simulink model "architecture1_copy"  (R2019b)
settings: Solver=VariableStepAuto  StartTime=0.0  StopTime=25000  RelTol=1e-3
undefined symbols (not defined in the file or in its folder): t_vect
libraries: xbsIndex_r4 x1103
settings Model: Creator=s4533087  LastModifiedBy=s4533087

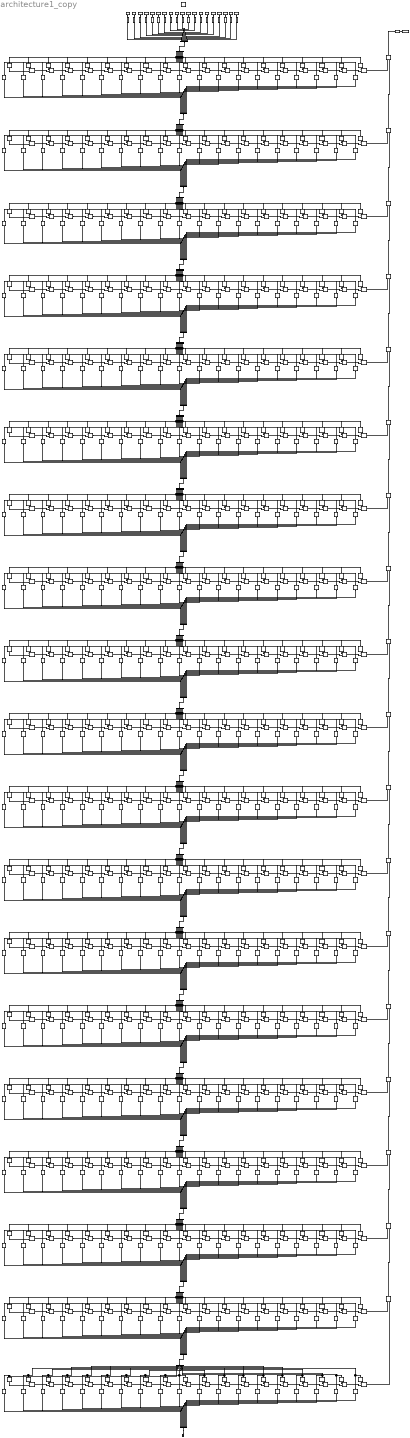
== system architecture1_copy ==
  note: Subsystem18
  note: Subsystem17
  note: Subsystem16
  note: Subsystem15
  note: Subsystem14
  note: Subsystem13
  note: Subsystem12
  note: Subsystem11
  note: Subsystem10
  note: Subsystem9
  note: Subsystem8
  note: Subsystem7
  note: Subsystem6
  note: Subsystem5
  note: Subsystem4
  note: Subsystem3
  note: Subsystem2
  note: Subsystem1
  note: Subsystem
  " System Generator" : xbsIndex_r4/ System Generator  Tag=genX  xilinxfamily=virtex7  part=xc7v2000t  speed=-1  package=flg1925  synthesis_tool=Vivado  clock_wrapper=Clock Enables  directory=./netlist  proj_type=Vivado  Synth_file=Vivado Synthesis Defaults  Impl_file=Vivado Implementation Defaults  testbench=off  simulink_period=1  sysclk_period=10  dcm_input_clock_period=10  incr_netlist=off  trim_vbits=Everywhere in SubSystem  dbl_ovrd=According to Block Masks  core_generation=According to Block Masks  run_coregen=off  deprecated_control=off  eval_field=0  block_type=sysgen
  AddSub{1..353,367,401,410,458,522,565,602} (360 alike) : xbsIndex_r4/AddSub  mode=Addition  use_carryin=off  use_carryout=off  en=off  latency=0  precision=Full  arith_type=Unsigned  n_bits=16  bin_pt=14  quantization=Truncate  overflow=Wrap  use_behavioral_HDL=off  hw_selection=Fabric  pipelined=off  dbl_ovrd=off  block_type=addsub
  Bus Creator{,1..19} (20 alike) : BusCreator  Inputs=19
  Bus Selector{,1..18} (19 alike) : BusSelector  OutputSignals=signal1,signal2,signal3,signal4,signal5,signal6,signal7,signal8,signal9,signal10,signal11,signal12,signal13,signal14,signal15,signal16,signal17,signal18,signal19
  CMult{,1,20,40,59,79,98,118,137,157,176,196,215,235,254,274,294,313,333} (19 alike) : xbsIndex_r4/CMult  const=t_vect(1)  gui_display_data_type=Fixed-point  const_n_bits=16  const_bin_pt=14  float_type=Single  exp_bits=8  fraction_bits=24  en=off  latency=0  precision=User Defined  arith_type="Signed  (2's comp)"  n_bits=Wc  bin_pt=Dc  quantization=Truncate  overflow=Flag as error  use_behavioral_HDL=off  mem_type=Distributed RAM  pipeline=off  dbl_ovrd=off  block_type=cmult
  CMult{10,29,49,68,88,107,127,146,166,186,205,225,244,264,283,303,323,342,360} (19 alike) : xbsIndex_r4/CMult  const=t_vect(12)  gui_display_data_type=Fixed-point  const_n_bits=16  const_bin_pt=14  float_type=Single  exp_bits=8  fraction_bits=24  en=off  latency=0  precision=User Defined  arith_type="Signed  (2's comp)"  n_bits=Wc  bin_pt=Dc  quantization=Truncate  overflow=Flag as error  use_behavioral_HDL=off  mem_type=Distributed RAM  pipeline=off  dbl_ovrd=off  block_type=cmult
  CMult{3,22,42,61,81,100,120,139,150,159,178,198,217,237,256,276,296,315,335} (19 alike) : xbsIndex_r4/CMult  const=t_vect(6)  gui_display_data_type=Fixed-point  const_n_bits=16  const_bin_pt=14  float_type=Single  exp_bits=8  fraction_bits=24  en=off  latency=0  precision=User Defined  arith_type="Signed  (2's comp)"  n_bits=Wc  bin_pt=Dc  quantization=Truncate  overflow=Flag as error  use_behavioral_HDL=off  mem_type=Distributed RAM  pipeline=off  dbl_ovrd=off  block_type=cmult
  CMult{4,23,43,62,82,101,121,140,160,179..180,199,218,238,257,277,297,316,336} (19 alike) : xbsIndex_r4/CMult  const=t_vect(5)  gui_display_data_type=Fixed-point  const_n_bits=16  const_bin_pt=14  float_type=Single  exp_bits=8  fraction_bits=24  en=off  latency=0  precision=User Defined  arith_type="Signed  (2's comp)"  n_bits=Wc  bin_pt=Dc  quantization=Truncate  overflow=Flag as error  use_behavioral_HDL=off  mem_type=Distributed RAM  pipeline=off  dbl_ovrd=off  block_type=cmult
  CMult{5,24,44,63,83,102,122,141,161,181,200,219..220,239,258,278,298,317,337} (19 alike) : xbsIndex_r4/CMult  const=t_vect(8)  gui_display_data_type=Fixed-point  const_n_bits=16  const_bin_pt=14  float_type=Single  exp_bits=8  fraction_bits=24  en=off  latency=0  precision=User Defined  arith_type="Signed  (2's comp)"  n_bits=Wc  bin_pt=Dc  quantization=Truncate  overflow=Flag as error  use_behavioral_HDL=off  mem_type=Distributed RAM  pipeline=off  dbl_ovrd=off  block_type=cmult
  CMult{6,25,45,64,84,103,123,142,162,182,201,221,240,259..260,279,299,318,338} (19 alike) : xbsIndex_r4/CMult  const=t_vect(10)  gui_display_data_type=Fixed-point  const_n_bits=16  const_bin_pt=14  float_type=Single  exp_bits=8  fraction_bits=24  en=off  latency=0  precision=User Defined  arith_type="Signed  (2's comp)"  n_bits=Wc  bin_pt=Dc  quantization=Truncate  overflow=Flag as error  use_behavioral_HDL=off  mem_type=Distributed RAM  pipeline=off  dbl_ovrd=off  block_type=cmult
  CMult{7,26,46,65,85,104,124,143,163,183,202,222,241,261,280,290,300,319,339} (19 alike) : xbsIndex_r4/CMult  const=t_vect(9)  gui_display_data_type=Fixed-point  const_n_bits=16  const_bin_pt=14  float_type=Single  exp_bits=8  fraction_bits=24  en=off  latency=0  precision=User Defined  arith_type="Signed  (2's comp)"  n_bits=Wc  bin_pt=Dc  quantization=Truncate  overflow=Flag as error  use_behavioral_HDL=off  mem_type=Distributed RAM  pipeline=off  dbl_ovrd=off  block_type=cmult
  CMult{8,27,47,66,86,105,125,144,164,184,203,223,242,262,281,301,320..321,340} (19 alike) : xbsIndex_r4/CMult  const=t_vect(7)  gui_display_data_type=Fixed-point  const_n_bits=16  const_bin_pt=14  float_type=Single  exp_bits=8  fraction_bits=24  en=off  latency=0  precision=User Defined  arith_type="Signed  (2's comp)"  n_bits=Wc  bin_pt=Dc  quantization=Truncate  overflow=Flag as error  use_behavioral_HDL=off  mem_type=Distributed RAM  pipeline=off  dbl_ovrd=off  block_type=cmult
  CMult{9,28,35,48,67,87,106,126,145,165,185,204,224,243,263,282,302,322,341} (19 alike) : xbsIndex_r4/CMult  const=t_vect(2)  gui_display_data_type=Fixed-point  const_n_bits=16  const_bin_pt=14  float_type=Single  exp_bits=8  fraction_bits=24  en=off  latency=0  precision=User Defined  arith_type="Signed  (2's comp)"  n_bits=Wc  bin_pt=Dc  quantization=Truncate  overflow=Flag as error  use_behavioral_HDL=off  mem_type=Distributed RAM  pipeline=off  dbl_ovrd=off  block_type=cmult
  CMult{11,30,50,69,89,108,128,147,167,187,206,226,245,265,284,304,324,343,400} (19 alike) : xbsIndex_r4/CMult  const=t_vect(14)  gui_display_data_type=Fixed-point  const_n_bits=16  const_bin_pt=14  float_type=Single  exp_bits=8  fraction_bits=24  en=off  latency=0  precision=User Defined  arith_type="Signed  (2's comp)"  n_bits=Wc  bin_pt=Dc  quantization=Truncate  overflow=Flag as error  use_behavioral_HDL=off  mem_type=Distributed RAM  pipeline=off  dbl_ovrd=off  block_type=cmult
  CMult{12,31,51,71,90,109,129,148,168,188,207,227,246,266,285,305,325,344,430} (19 alike) : xbsIndex_r4/CMult  const=t_vect(13)  gui_display_data_type=Fixed-point  const_n_bits=16  const_bin_pt=14  float_type=Single  exp_bits=8  fraction_bits=24  en=off  latency=0  precision=User Defined  arith_type="Signed  (2's comp)"  n_bits=Wc  bin_pt=Dc  quantization=Truncate  overflow=Flag as error  use_behavioral_HDL=off  mem_type=Distributed RAM  pipeline=off  dbl_ovrd=off  block_type=cmult
  CMult{2,21,41,60,80,99,110,119,138,158,177,197,216,236,255,275,295,314,334} (19 alike) : xbsIndex_r4/CMult  const=t_vect(4)  gui_display_data_type=Fixed-point  const_n_bits=16  const_bin_pt=14  float_type=Single  exp_bits=8  fraction_bits=24  en=off  latency=0  precision=User Defined  arith_type="Signed  (2's comp)"  n_bits=Wc  bin_pt=Dc  quantization=Truncate  overflow=Flag as error  use_behavioral_HDL=off  mem_type=Distributed RAM  pipeline=off  dbl_ovrd=off  block_type=cmult
  CMult{13,32,52,72,91,111,130,149,169,189,208,228,247,267,286,306,326,345,470} (19 alike) : xbsIndex_r4/CMult  const=t_vect(16)  gui_display_data_type=Fixed-point  const_n_bits=16  const_bin_pt=14  float_type=Single  exp_bits=8  fraction_bits=24  en=off  latency=0  precision=User Defined  arith_type="Signed  (2's comp)"  n_bits=Wc  bin_pt=Dc  quantization=Truncate  overflow=Flag as error  use_behavioral_HDL=off  mem_type=Distributed RAM  pipeline=off  dbl_ovrd=off  block_type=cmult
  CMult{14,33,53,73,92,112,131,151,170,190,209,229,248,268,287,307,327,346,510} (19 alike) : xbsIndex_r4/CMult  const=t_vect(18)  gui_display_data_type=Fixed-point  const_n_bits=16  const_bin_pt=14  float_type=Single  exp_bits=8  fraction_bits=24  en=off  latency=0  precision=User Defined  arith_type="Signed  (2's comp)"  n_bits=Wc  bin_pt=Dc  quantization=Truncate  overflow=Flag as error  use_behavioral_HDL=off  mem_type=Distributed RAM  pipeline=off  dbl_ovrd=off  block_type=cmult
  CMult{15,34,54,74,93,113,132,152,171,191,210,230,249,269,288,308,328,347,540} (19 alike) : xbsIndex_r4/CMult  const=t_vect(17)  gui_display_data_type=Fixed-point  const_n_bits=16  const_bin_pt=14  float_type=Single  exp_bits=8  fraction_bits=24  en=off  latency=0  precision=User Defined  arith_type="Signed  (2's comp)"  n_bits=Wc  bin_pt=Dc  quantization=Truncate  overflow=Flag as error  use_behavioral_HDL=off  mem_type=Distributed RAM  pipeline=off  dbl_ovrd=off  block_type=cmult
  CMult{16,36,55,75,94,114,133,153,172,192,211,231,250,270,289,309,329,348,570} (19 alike) : xbsIndex_r4/CMult  const=t_vect(15)  gui_display_data_type=Fixed-point  const_n_bits=16  const_bin_pt=14  float_type=Single  exp_bits=8  fraction_bits=24  en=off  latency=0  precision=User Defined  arith_type="Signed  (2's comp)"  n_bits=Wc  bin_pt=Dc  quantization=Truncate  overflow=Flag as error  use_behavioral_HDL=off  mem_type=Distributed RAM  pipeline=off  dbl_ovrd=off  block_type=cmult
  CMult{17,37,56,76,95,115,134,154,173,193,212,232,251,271,291,310,330,349,600} (19 alike) : xbsIndex_r4/CMult  const=t_vect(11)  gui_display_data_type=Fixed-point  const_n_bits=16  const_bin_pt=14  float_type=Single  exp_bits=8  fraction_bits=24  en=off  latency=0  precision=User Defined  arith_type="Signed  (2's comp)"  n_bits=Wc  bin_pt=Dc  quantization=Truncate  overflow=Flag as error  use_behavioral_HDL=off  mem_type=Distributed RAM  pipeline=off  dbl_ovrd=off  block_type=cmult
  CMult{18,38,57,77,96,116,135,155,174,194,213,233,252,272,292,311,331,350,635} (19 alike) : xbsIndex_r4/CMult  const=t_vect(19)  gui_display_data_type=Fixed-point  const_n_bits=16  const_bin_pt=14  float_type=Single  exp_bits=8  fraction_bits=24  en=off  latency=0  precision=User Defined  arith_type="Signed  (2's comp)"  n_bits=Wc  bin_pt=Dc  quantization=Truncate  overflow=Flag as error  use_behavioral_HDL=off  mem_type=Distributed RAM  pipeline=off  dbl_ovrd=off  block_type=cmult
  CMult{19,39,58,70,78,97,117,136,156,175,195,214,234,253,273,293,312,332,351} (19 alike) : xbsIndex_r4/CMult  const=t_vect(3)  gui_display_data_type=Fixed-point  const_n_bits=16  const_bin_pt=14  float_type=Single  exp_bits=8  fraction_bits=24  en=off  latency=0  precision=User Defined  arith_type="Signed  (2's comp)"  n_bits=Wc  bin_pt=Dc  quantization=Truncate  overflow=Flag as error  use_behavioral_HDL=off  mem_type=Distributed RAM  pipeline=off  dbl_ovrd=off  block_type=cmult
  Delay{,1..352,380,412,448,484,516,548,580,614} (361 alike) : xbsIndex_r4/Delay  rst=off  infoeditControl=Selection of Reset will increase slice count due to use of real FFs and instead of SRLs  en=off  latency=1  reg_retiming=off  dbl_ovrd=off  block_type=delay
  From Workspace : FromWorkspace  VariableName=[(1:1:length(sig(:, 1)))' sig(:, 1)]  SampleTime=0
  From Workspace1 : FromWorkspace  VariableName=[(1:1:length(sig(:, 2)))' sig(:, 2)];  SampleTime=0
  From Workspace10 : FromWorkspace  VariableName=[(1:1:length(sig(:, 11)))' sig(:, 11)];  SampleTime=0
  From Workspace11 : FromWorkspace  VariableName=[(1:1:length(sig(:, 12)))' sig(:, 12)];  SampleTime=0
  From Workspace12 : FromWorkspace  VariableName=[(1:1:length(sig(:, 13)))' sig(:, 13)];  SampleTime=0
  From Workspace13 : FromWorkspace  VariableName=[(1:1:length(sig(:, 14)))' sig(:, 14)];  SampleTime=0
  From Workspace14 : FromWorkspace  VariableName=[(1:1:length(sig(:, 15)))' sig(:, 15)];  SampleTime=0
  From Workspace15 : FromWorkspace  VariableName=[(1:1:length(sig(:, 16)))' sig(:, 16)];  SampleTime=0
  From Workspace16 : FromWorkspace  VariableName=[(1:1:length(sig(:, 17)))' sig(:, 17)];  SampleTime=0
  From Workspace17 : FromWorkspace  VariableName=[(1:1:length(sig(:, 18)))' sig(:, 18)];  SampleTime=0
  From Workspace18 : FromWorkspace  VariableName=[(1:1:length(sig(:, 19)))' sig(:, 19)];  SampleTime=0
  From Workspace2 : FromWorkspace  VariableName=[(1:1:length(sig(:, 3)))' sig(:, 3)];  SampleTime=0
  From Workspace3 : FromWorkspace  VariableName=[(1:1:length(sig(:, 4)))' sig(:, 4)];  SampleTime=0
  From Workspace4 : FromWorkspace  VariableName=[(1:1:length(sig(:, 5)))' sig(:, 5)];  SampleTime=0
  From Workspace5 : FromWorkspace  VariableName=[(1:1:length(sig(:, 6)))' sig(:, 6)];  SampleTime=0
  From Workspace6 : FromWorkspace  VariableName=[(1:1:length(sig(:, 7)))' sig(:, 7)];  SampleTime=0
  From Workspace7 : FromWorkspace  VariableName=[(1:1:length(sig(:, 8)))' sig(:, 8)];  SampleTime=0
  From Workspace8 : FromWorkspace  VariableName=[(1:1:length(sig(:, 9)))' sig(:, 9)];  SampleTime=0
  From Workspace9 : FromWorkspace  VariableName=[(1:1:length(sig(:, 10)))' sig(:, 10)];  SampleTime=0
  Gateway In{27,36..45,47,57,64..69} (19 alike) : xbsIndex_r4/Gateway In  gui_display_data_type=Fixed-point  arith_type="Signed  (2's comp)"  n_bits=W  bin_pt=D  preci_type=Single  exp_width=8  frac_width=24  rows=1  columns=1  quantization="Round  (unbiased: +/- Inf)"  overflow=Saturate  period=1  UseAsADC=off  ADCChannel='1'  interface=None  automatic_assignment=on  address_offset=hex2dec('00')  intf_name=''  intf_description=''  default_value=0  timing_constraint=None  locs_specified=off  LOCs={}  io_standard={}  inherit_from_input=off  hdl_port=on  dbl_ovrd=off  block_type=gatewayin
  Gateway Out1 : xbsIndex_r4/Gateway Out  inherit_from_input=off  hdl_port=on  rows=1  columns=1  UseAsDAC=off  DACChannel='1'  interface=None  automatic_assignment=on  address_offset=hex2dec('00')  intf_name=''  intf_description=''  timing_constraint=None  locs_specified=off  LOCs={}  io_standard={}  block_type=gatewayout
  Terminator : Terminator
  To Workspace1 : ToWorkspace  VariableName=C  SaveFormat=Timeseries  SampleTime=-1
  wires:
  Gateway Out1/1 -> To Workspace1/1
  From Workspace/1 -> Gateway In27/1
  From Workspace1/1 -> Gateway In36/1
  From Workspace2/1 -> Gateway In47/1
  From Workspace3/1 -> Gateway In57/1
  From Workspace4/1 -> Gateway In64/1
  From Workspace5/1 -> Gateway In65/1
  From Workspace6/1 -> Gateway In66/1
  From Workspace7/1 -> Gateway In67/1
  From Workspace8/1 -> Gateway In68/1
  From Workspace9/1 -> Gateway In69/1
  From Workspace10/1 -> Gateway In37/1
  From Workspace11/1 -> Gateway In38/1
  From Workspace12/1 -> Gateway In39/1
  From Workspace13/1 -> Gateway In40/1
  From Workspace14/1 -> Gateway In41/1
  From Workspace15/1 -> Gateway In42/1
  From Workspace16/1 -> Gateway In43/1
  From Workspace17/1 -> Gateway In44/1
  From Workspace18/1 -> Gateway In45/1
  Gateway In36/1 -> Bus Creator/2
  Gateway In47/1 -> Bus Creator/3
  Gateway In57/1 -> Bus Creator/4
  Gateway In64/1 -> Bus Creator/5
  Gateway In65/1 -> Bus Creator/6
  Gateway In66/1 -> Bus Creator/7
  Gateway In67/1 -> Bus Creator/8
  Gateway In68/1 -> Bus Creator/9
  Gateway In69/1 -> Bus Creator/10
  Gateway In37/1 -> Bus Creator/11
  Gateway In38/1 -> Bus Creator/12
  Gateway In39/1 -> Bus Creator/13
  Gateway In40/1 -> Bus Creator/14
  Gateway In41/1 -> Bus Creator/15
  Gateway In42/1 -> Bus Creator/16
  Gateway In43/1 -> Bus Creator/17
  Gateway In44/1 -> Bus Creator/18
  Gateway In45/1 -> Bus Creator/19
  Gateway In27/1 -> Bus Creator/1
  AddSub602/1 -> AddSub26/1
  AddSub26/1 -> Gateway Out1/1
  AddSub37/1 -> AddSub1/1
  AddSub55/1 -> AddSub2/1
  AddSub74/1 -> AddSub3/1
  AddSub92/1 -> AddSub6/1
  AddSub111/1 -> AddSub4/1
  AddSub129/1 -> AddSub5/1
  AddSub148/1 -> AddSub7/1
  AddSub186/1 -> AddSub8/1
  AddSub259/1 -> AddSub12/1
  AddSub166/1 -> AddSub10/1
  AddSub204/1 -> AddSub9/1
  AddSub277/1 -> AddSub13/1
  AddSub222/1 -> AddSub11/1
  AddSub296/1 -> AddSub15/1
  AddSub241/1 -> AddSub14/1
  AddSub334/1 -> AddSub16/1
  AddSub314/1 -> AddSub18/1
  AddSub352/1 -> AddSub16/2
  AddSub16/1 -> AddSub18/2
  AddSub18/1 -> AddSub15/2
  AddSub15/1 -> AddSub13/2
  AddSub13/1 -> AddSub12/2
  AddSub12/1 -> AddSub14/2
  AddSub14/1 -> AddSub11/2
  AddSub11/1 -> AddSub9/2
  AddSub9/1 -> AddSub8/2
  AddSub8/1 -> AddSub10/2
  AddSub10/1 -> AddSub7/2
  AddSub7/1 -> AddSub5/2
  AddSub5/1 -> AddSub4/2
  AddSub4/1 -> AddSub6/2
  AddSub6/1 -> AddSub3/2
  AddSub3/1 -> AddSub2/2
  AddSub2/1 -> AddSub1/2
  AddSub1/1 -> AddSub26/2
  Bus Creator19/1 -> Terminator/1
  CMult180/1 -> AddSub106/1
  Delay448/1 -> Bus Creator1/16
  Delay34/1 -> Bus Creator1/2
  AddSub367/1 -> AddSub401/2
  AddSub458/1 -> AddSub602/2
  CMult570/1 -> AddSub401/1
  Bus Selector/7 -> Delay308/1, CMult320/1  "<signal7>"
  Bus Creator/1 -> Bus Selector/1
  AddSub145/1 -> AddSub176/2
  Delay548/1 -> Bus Creator1/15
  CMult290/1 -> AddSub184/1
  AddSub17/1 -> AddSub71/2
  Delay308/1 -> Bus Creator1/7
  Delay208/1 -> Bus Creator1/8
  CMult540/1 -> AddSub410/1
  AddSub316/1 -> AddSub565/2
  Delay68/1 -> Bus Creator1/3
  Bus Selector/2 -> Delay34/1, CMult35/1  "<signal2>"
  CMult510/1 -> AddSub458/1
  Delay/1 -> Bus Creator1/1
  CMult70/1 -> AddSub17/1
  Bus Selector/19 -> CMult635/1, Delay614/1  "<signal19>"
  Delay172/1 -> Bus Creator1/5
  AddSub35/1 -> AddSub17/2
  AddSub410/1 -> AddSub458/2
  Bus Selector/13 -> CMult430/1, Delay412/1  "<signal13>"
  Bus Selector/10 -> CMult260/1, Delay244/1  "<signal10>"
  CMult600/1 -> AddSub316/1
  AddSub227/1 -> AddSub316/2
  CMult360/1 -> AddSub565/1
  CMult320/1 -> AddSub176/1
  Delay344/1 -> Bus Creator1/12
  Delay380/1 -> Bus Creator1/14
  Bus Selector/12 -> CMult360/1, Delay344/1  "<signal12>"
  CMult470/1 -> AddSub522/1
  Delay484/1 -> Bus Creator1/18
  Bus Selector/15 -> CMult570/1, Delay548/1  "<signal15>"
  Bus Selector/9 -> Delay276/1, CMult290/1  "<signal9>"
  AddSub565/1 -> AddSub324/2
  Delay412/1 -> Bus Creator1/13
  Delay244/1 -> Bus Creator1/10
  Bus Selector/17 -> CMult540/1, Delay516/1  "<signal17>"
  Delay140/1 -> Bus Creator1/6
  AddSub285/1 -> AddSub184/2
  Delay516/1 -> Bus Creator1/17
  Delay580/1 -> Bus Creator1/11
  Bus Selector/14 -> CMult400/1, Delay380/1  "<signal14>"
  CMult110/1 -> AddSub71/1
  AddSub184/1 -> AddSub227/2
  Bus Selector/16 -> CMult470/1, Delay448/1  "<signal16>"
  Bus Selector/3 -> Delay68/1, CMult70/1  "<signal3>"
  AddSub176/1 -> AddSub285/2
  Bus Selector/8 -> Delay208/1, CMult220/1  "<signal8>"
  CMult35/1 -> AddSub35/1
  CMult400/1 -> AddSub367/1
  Bus Selector/1 -> Delay/1, CMult/1  "<signal1>"
  Bus Selector/6 -> Delay140/1, CMult150/1  "<signal6>"
  CMult635/1 -> AddSub602/1
  Bus Selector/18 -> CMult510/1, Delay484/1  "<signal18>"
  CMult260/1 -> AddSub227/1
  Bus Selector/4 -> Delay104/1, CMult110/1  "<signal4>"
  AddSub324/1 -> AddSub367/2
  Delay276/1 -> Bus Creator1/9
  CMult150/1 -> AddSub145/1
  AddSub71/1 -> AddSub106/2
  Delay104/1 -> Bus Creator1/4
  AddSub522/1 -> AddSub410/2
  Delay614/1 -> Bus Creator1/19
  Bus Selector/5 -> Delay172/1, CMult180/1  "<signal5>"
  CMult/1 -> AddSub35/2
  CMult430/1 -> AddSub324/1
  AddSub401/1 -> AddSub522/2
  CMult220/1 -> AddSub285/1
  AddSub106/1 -> AddSub145/2
  Bus Selector/11 -> CMult600/1, Delay580/1  "<signal11>"
  CMult4/1 -> AddSub20/1
  Delay13/1 -> Bus Creator2/16
  Delay9/1 -> Bus Creator2/2
  AddSub30/1 -> AddSub31/2
  AddSub33/1 -> AddSub37/2
  CMult16/1 -> AddSub31/1
  Bus Selector1/7 -> Delay8/1, CMult8/1  "<signal7>"
  Bus Creator1/1 -> Bus Selector1/1
  AddSub21/1 -> AddSub22/2
  Delay16/1 -> Bus Creator2/15
  CMult7/1 -> AddSub23/1
  AddSub19/1 -> AddSub38/2
  Delay8/1 -> Bus Creator2/7
  Delay5/1 -> Bus Creator2/8
  CMult15/1 -> AddSub32/1
  AddSub27/1 -> AddSub36/2
  Delay19/1 -> Bus Creator2/3
  Bus Selector1/2 -> Delay9/1, CMult9/1  "<signal2>"
  CMult14/1 -> AddSub33/1
  Delay1/1 -> Bus Creator2/1
  CMult19/1 -> AddSub19/1
  Bus Selector1/19 -> CMult18/1, Delay18/1  "<signal19>"
  Delay4/1 -> Bus Creator2/5
  AddSub29/1 -> AddSub19/2
  AddSub32/1 -> AddSub33/2
  Bus Selector1/13 -> CMult12/1, Delay12/1  "<signal13>"
  Bus Selector1/10 -> CMult6/1, Delay6/1  "<signal10>"
  CMult17/1 -> AddSub27/1
  AddSub24/1 -> AddSub27/2
  CMult10/1 -> AddSub36/1
  CMult8/1 -> AddSub22/1
  Delay10/1 -> Bus Creator2/12
  Delay11/1 -> Bus Creator2/14
  Bus Selector1/12 -> CMult10/1, Delay10/1  "<signal12>"
  CMult13/1 -> AddSub34/1
  Delay14/1 -> Bus Creator2/18
  Bus Selector1/15 -> CMult16/1, Delay16/1  "<signal15>"
  Bus Selector1/9 -> Delay7/1, CMult7/1  "<signal9>"
  AddSub36/1 -> AddSub28/2
  Delay12/1 -> Bus Creator2/13
  Delay6/1 -> Bus Creator2/10
  Bus Selector1/17 -> CMult15/1, Delay15/1  "<signal17>"
  Delay3/1 -> Bus Creator2/6
  AddSub25/1 -> AddSub23/2
  Delay15/1 -> Bus Creator2/17
  Delay17/1 -> Bus Creator2/11
  Bus Selector1/14 -> CMult11/1, Delay11/1  "<signal14>"
  CMult2/1 -> AddSub38/1
  AddSub23/1 -> AddSub24/2
  Bus Selector1/16 -> CMult13/1, Delay13/1  "<signal16>"
  Bus Selector1/3 -> Delay19/1, CMult19/1  "<signal3>"
  AddSub22/1 -> AddSub25/2
  Bus Selector1/8 -> Delay5/1, CMult5/1  "<signal8>"
  CMult9/1 -> AddSub29/1
  CMult11/1 -> AddSub30/1
  Bus Selector1/1 -> Delay1/1, CMult1/1  "<signal1>"
  Bus Selector1/6 -> Delay3/1, CMult3/1  "<signal6>"
  CMult18/1 -> AddSub37/1
  Bus Selector1/18 -> CMult14/1, Delay14/1  "<signal18>"
  CMult6/1 -> AddSub24/1
  Bus Selector1/4 -> Delay2/1, CMult2/1  "<signal4>"
  AddSub28/1 -> AddSub30/2
  Delay7/1 -> Bus Creator2/9
  CMult3/1 -> AddSub21/1
  AddSub38/1 -> AddSub20/2
  Delay2/1 -> Bus Creator2/4
  AddSub34/1 -> AddSub32/2
  Delay18/1 -> Bus Creator2/19
  Bus Selector1/5 -> Delay4/1, CMult4/1  "<signal5>"
  CMult1/1 -> AddSub29/2
  CMult12/1 -> AddSub28/1
  AddSub31/1 -> AddSub34/2
  CMult5/1 -> AddSub25/1
  AddSub20/1 -> AddSub21/2
  Bus Selector1/11 -> CMult17/1, Delay17/1  "<signal11>"
  CMult23/1 -> AddSub40/1
  Delay32/1 -> Bus Creator3/16
  Delay28/1 -> Bus Creator3/2
  AddSub49/1 -> AddSub50/2
  AddSub52/1 -> AddSub55/2
  CMult36/1 -> AddSub50/1
  Bus Selector2/7 -> Delay27/1, CMult27/1  "<signal7>"
  Bus Creator2/1 -> Bus Selector2/1
  AddSub41/1 -> AddSub42/2
  Delay36/1 -> Bus Creator3/15
  CMult26/1 -> AddSub43/1
  AddSub39/1 -> AddSub56/2
  Delay27/1 -> Bus Creator3/7
  Delay24/1 -> Bus Creator3/8
  CMult34/1 -> AddSub51/1
  AddSub46/1 -> AddSub54/2
  Delay39/1 -> Bus Creator3/3
  Bus Selector2/2 -> Delay28/1, CMult28/1  "<signal2>"
  CMult33/1 -> AddSub52/1
  Delay20/1 -> Bus Creator3/1
  CMult39/1 -> AddSub39/1
  Bus Selector2/19 -> CMult38/1, Delay38/1  "<signal19>"
  Delay23/1 -> Bus Creator3/5
  AddSub48/1 -> AddSub39/2
  AddSub51/1 -> AddSub52/2
  Bus Selector2/13 -> Delay31/1, CMult31/1  "<signal13>"
  Bus Selector2/10 -> CMult25/1, Delay25/1  "<signal10>"
  CMult37/1 -> AddSub46/1
  AddSub44/1 -> AddSub46/2
  CMult29/1 -> AddSub54/1
  CMult27/1 -> AddSub42/1
  Delay29/1 -> Bus Creator3/12
  Delay30/1 -> Bus Creator3/14
  Bus Selector2/12 -> Delay29/1, CMult29/1  "<signal12>"
  CMult32/1 -> AddSub53/1
  Delay33/1 -> Bus Creator3/18
  Bus Selector2/15 -> Delay36/1, CMult36/1  "<signal15>"
  Bus Selector2/9 -> Delay26/1, CMult26/1  "<signal9>"
  AddSub54/1 -> AddSub47/2
  Delay31/1 -> Bus Creator3/13
  Delay25/1 -> Bus Creator3/10
  Bus Selector2/17 -> Delay35/1, CMult34/1  "<signal17>"
  Delay22/1 -> Bus Creator3/6
  AddSub45/1 -> AddSub43/2
  Delay35/1 -> Bus Creator3/17
  Delay37/1 -> Bus Creator3/11
  Bus Selector2/14 -> Delay30/1, CMult30/1  "<signal14>"
  CMult21/1 -> AddSub56/1
  AddSub43/1 -> AddSub44/2
  Bus Selector2/16 -> Delay32/1, CMult32/1  "<signal16>"
  Bus Selector2/3 -> Delay39/1, CMult39/1  "<signal3>"
  AddSub42/1 -> AddSub45/2
  Bus Selector2/8 -> Delay24/1, CMult24/1  "<signal8>"
  CMult28/1 -> AddSub48/1
  CMult30/1 -> AddSub49/1
  Bus Selector2/1 -> Delay20/1, CMult20/1  "<signal1>"
  Bus Selector2/6 -> Delay22/1, CMult22/1  "<signal6>"
  CMult38/1 -> AddSub55/1
  Bus Selector2/18 -> CMult33/1, Delay33/1  "<signal18>"
  CMult25/1 -> AddSub44/1
  Bus Selector2/4 -> Delay21/1, CMult21/1  "<signal4>"
  AddSub47/1 -> AddSub49/2
  Delay26/1 -> Bus Creator3/9
  CMult22/1 -> AddSub41/1
  AddSub56/1 -> AddSub40/2
  Delay21/1 -> Bus Creator3/4
  AddSub53/1 -> AddSub51/2
  Delay38/1 -> Bus Creator3/19
  Bus Selector2/5 -> Delay23/1, CMult23/1  "<signal5>"
  CMult20/1 -> AddSub48/2
  CMult31/1 -> AddSub47/1
  AddSub50/1 -> AddSub53/2
  CMult24/1 -> AddSub45/1
  AddSub40/1 -> AddSub41/2
  Bus Selector2/11 -> Delay37/1, CMult37/1  "<signal11>"
  CMult43/1 -> AddSub58/1
  Delay52/1 -> Bus Creator4/16
  Delay48/1 -> Bus Creator4/2
  AddSub67/1 -> AddSub68/2
  AddSub70/1 -> AddSub74/2
  CMult55/1 -> AddSub68/1
  Bus Selector3/7 -> Delay47/1, CMult47/1  "<signal7>"
  Bus Creator3/1 -> Bus Selector3/1
  AddSub59/1 -> AddSub60/2
  Delay55/1 -> Bus Creator4/15
  CMult46/1 -> AddSub61/1
  AddSub57/1 -> AddSub75/2
  Delay47/1 -> Bus Creator4/7
  Delay44/1 -> Bus Creator4/8
  CMult54/1 -> AddSub69/1
  AddSub64/1 -> AddSub73/2
  Delay58/1 -> Bus Creator4/3
  Bus Selector3/2 -> Delay48/1, CMult48/1  "<signal2>"
  CMult53/1 -> AddSub70/1
  Delay40/1 -> Bus Creator4/1
  CMult58/1 -> AddSub57/1
  Bus Selector3/19 -> CMult57/1, Delay57/1  "<signal19>"
  Delay43/1 -> Bus Creator4/5
  AddSub66/1 -> AddSub57/2
  AddSub69/1 -> AddSub70/2
  Bus Selector3/13 -> Delay51/1, CMult51/1  "<signal13>"
  Bus Selector3/10 -> CMult45/1, Delay45/1  "<signal10>"
  CMult56/1 -> AddSub64/1
  AddSub62/1 -> AddSub64/2
  CMult49/1 -> AddSub73/1
  CMult47/1 -> AddSub60/1
  Delay49/1 -> Bus Creator4/12
  Delay50/1 -> Bus Creator4/14
  Bus Selector3/12 -> Delay49/1, CMult49/1  "<signal12>"
  CMult52/1 -> AddSub72/1
  Delay53/1 -> Bus Creator4/18
  Bus Selector3/15 -> Delay55/1, CMult55/1  "<signal15>"
  Bus Selector3/9 -> Delay46/1, CMult46/1  "<signal9>"
  AddSub73/1 -> AddSub65/2
  Delay51/1 -> Bus Creator4/13
  Delay45/1 -> Bus Creator4/10
  Bus Selector3/17 -> Delay54/1, CMult54/1  "<signal17>"
  Delay42/1 -> Bus Creator4/6
  AddSub63/1 -> AddSub61/2
  Delay54/1 -> Bus Creator4/17
  Delay56/1 -> Bus Creator4/11
  Bus Selector3/14 -> Delay50/1, CMult50/1  "<signal14>"
  CMult41/1 -> AddSub75/1
  AddSub61/1 -> AddSub62/2
  Bus Selector3/16 -> Delay52/1, CMult52/1  "<signal16>"
  Bus Selector3/3 -> Delay58/1, CMult58/1  "<signal3>"
  AddSub60/1 -> AddSub63/2
  Bus Selector3/8 -> Delay44/1, CMult44/1  "<signal8>"
  CMult48/1 -> AddSub66/1
  CMult50/1 -> AddSub67/1
  Bus Selector3/1 -> Delay40/1, CMult40/1  "<signal1>"
  Bus Selector3/6 -> Delay42/1, CMult42/1  "<signal6>"
  CMult57/1 -> AddSub74/1
  Bus Selector3/18 -> CMult53/1, Delay53/1  "<signal18>"
  CMult45/1 -> AddSub62/1
  Bus Selector3/4 -> Delay41/1, CMult41/1  "<signal4>"
  AddSub65/1 -> AddSub67/2
  Delay46/1 -> Bus Creator4/9
  CMult42/1 -> AddSub59/1
  AddSub75/1 -> AddSub58/2
  Delay41/1 -> Bus Creator4/4
  AddSub72/1 -> AddSub69/2
  Delay57/1 -> Bus Creator4/19
  Bus Selector3/5 -> Delay43/1, CMult43/1  "<signal5>"
  CMult40/1 -> AddSub66/2
  CMult51/1 -> AddSub65/1
  AddSub68/1 -> AddSub72/2
  CMult44/1 -> AddSub63/1
  AddSub58/1 -> AddSub59/2
  Bus Selector3/11 -> Delay56/1, CMult56/1  "<signal11>"
  CMult62/1 -> AddSub77/1
  Delay72/1 -> Bus Creator5/16
  Delay67/1 -> Bus Creator5/2
  AddSub86/1 -> AddSub87/2
  AddSub89/1 -> AddSub92/2
  CMult75/1 -> AddSub87/1
  Bus Selector4/7 -> Delay66/1, CMult66/1  "<signal7>"
  Bus Creator4/1 -> Bus Selector4/1
  AddSub78/1 -> AddSub79/2
  Delay75/1 -> Bus Creator5/15
  CMult65/1 -> AddSub80/1
  AddSub76/1 -> AddSub93/2
  Delay66/1 -> Bus Creator5/7
  Delay63/1 -> Bus Creator5/8
  CMult74/1 -> AddSub88/1
  AddSub83/1 -> AddSub91/2
  Delay78/1 -> Bus Creator5/3
  Bus Selector4/2 -> Delay67/1, CMult67/1  "<signal2>"
  CMult73/1 -> AddSub89/1
  Delay59/1 -> Bus Creator5/1
  CMult78/1 -> AddSub76/1
  Bus Selector4/19 -> CMult77/1, Delay77/1  "<signal19>"
  Delay62/1 -> Bus Creator5/5
  AddSub85/1 -> AddSub76/2
  AddSub88/1 -> AddSub89/2
  Bus Selector4/13 -> Delay71/1, CMult71/1  "<signal13>"
  Bus Selector4/10 -> CMult64/1, Delay64/1  "<signal10>"
  CMult76/1 -> AddSub83/1
  AddSub81/1 -> AddSub83/2
  CMult68/1 -> AddSub91/1
  CMult66/1 -> AddSub79/1
  Delay69/1 -> Bus Creator5/12
  Delay70/1 -> Bus Creator5/14
  Bus Selector4/12 -> Delay69/1, CMult68/1  "<signal12>"
  CMult72/1 -> AddSub90/1
  Delay73/1 -> Bus Creator5/18
  Bus Selector4/15 -> Delay75/1, CMult75/1  "<signal15>"
  Bus Selector4/9 -> Delay65/1, CMult65/1  "<signal9>"
  AddSub91/1 -> AddSub84/2
  Delay71/1 -> Bus Creator5/13
  Delay64/1 -> Bus Creator5/10
  Bus Selector4/17 -> Delay74/1, CMult74/1  "<signal17>"
  Delay61/1 -> Bus Creator5/6
  AddSub82/1 -> AddSub80/2
  Delay74/1 -> Bus Creator5/17
  Delay76/1 -> Bus Creator5/11
  Bus Selector4/14 -> Delay70/1, CMult69/1  "<signal14>"
  CMult60/1 -> AddSub93/1
  AddSub80/1 -> AddSub81/2
  Bus Selector4/16 -> Delay72/1, CMult72/1  "<signal16>"
  Bus Selector4/3 -> Delay78/1, CMult78/1  "<signal3>"
  AddSub79/1 -> AddSub82/2
  Bus Selector4/8 -> Delay63/1, CMult63/1  "<signal8>"
  CMult67/1 -> AddSub85/1
  CMult69/1 -> AddSub86/1
  Bus Selector4/1 -> Delay59/1, CMult59/1  "<signal1>"
  Bus Selector4/6 -> Delay61/1, CMult61/1  "<signal6>"
  CMult77/1 -> AddSub92/1
  Bus Selector4/18 -> CMult73/1, Delay73/1  "<signal18>"
  CMult64/1 -> AddSub81/1
  Bus Selector4/4 -> Delay60/1, CMult60/1  "<signal4>"
  AddSub84/1 -> AddSub86/2
  Delay65/1 -> Bus Creator5/9
  CMult61/1 -> AddSub78/1
  AddSub93/1 -> AddSub77/2
  Delay60/1 -> Bus Creator5/4
  AddSub90/1 -> AddSub88/2
  Delay77/1 -> Bus Creator5/19
  Bus Selector4/5 -> Delay62/1, CMult62/1  "<signal5>"
  CMult59/1 -> AddSub85/2
  CMult71/1 -> AddSub84/1
  AddSub87/1 -> AddSub90/2
  CMult63/1 -> AddSub82/1
  AddSub77/1 -> AddSub78/2
  Bus Selector4/11 -> Delay76/1, CMult76/1  "<signal11>"
  CMult82/1 -> AddSub95/1
  Delay91/1 -> Bus Creator6/16
  Delay87/1 -> Bus Creator6/2
  AddSub104/1 -> AddSub105/2
  AddSub108/1 -> AddSub111/2
  CMult94/1 -> AddSub105/1
  Bus Selector5/7 -> Delay86/1, CMult86/1  "<signal7>"
  Bus Creator5/1 -> Bus Selector5/1
  AddSub96/1 -> AddSub97/2
  Delay94/1 -> Bus Creator6/15
  CMult85/1 -> AddSub98/1
  AddSub94/1 -> AddSub112/2
  Delay86/1 -> Bus Creator6/7
  Delay83/1 -> Bus Creator6/8
  CMult93/1 -> AddSub107/1
  AddSub101/1 -> AddSub110/2
  Delay97/1 -> Bus Creator6/3
  Bus Selector5/2 -> Delay87/1, CMult87/1  "<signal2>"
  CMult92/1 -> AddSub108/1
  Delay79/1 -> Bus Creator6/1
  CMult97/1 -> AddSub94/1
  Bus Selector5/19 -> CMult96/1, Delay96/1  "<signal19>"
  Delay82/1 -> Bus Creator6/5
  AddSub103/1 -> AddSub94/2
  AddSub107/1 -> AddSub108/2
  Bus Selector5/13 -> Delay90/1, CMult90/1  "<signal13>"
  Bus Selector5/10 -> CMult84/1, Delay84/1  "<signal10>"
  CMult95/1 -> AddSub101/1
  AddSub99/1 -> AddSub101/2
  CMult88/1 -> AddSub110/1
  CMult86/1 -> AddSub97/1
  Delay88/1 -> Bus Creator6/12
  Delay89/1 -> Bus Creator6/14
  Bus Selector5/12 -> Delay88/1, CMult88/1  "<signal12>"
  CMult91/1 -> AddSub109/1
  Delay92/1 -> Bus Creator6/18
  Bus Selector5/15 -> Delay94/1, CMult94/1  "<signal15>"
  Bus Selector5/9 -> Delay85/1, CMult85/1  "<signal9>"
  AddSub110/1 -> AddSub102/2
  Delay90/1 -> Bus Creator6/13
  Delay84/1 -> Bus Creator6/10
  Bus Selector5/17 -> Delay93/1, CMult93/1  "<signal17>"
  Delay81/1 -> Bus Creator6/6
  AddSub100/1 -> AddSub98/2
  Delay93/1 -> Bus Creator6/17
  Delay95/1 -> Bus Creator6/11
  Bus Selector5/14 -> Delay89/1, CMult89/1  "<signal14>"
  CMult80/1 -> AddSub112/1
  AddSub98/1 -> AddSub99/2
  Bus Selector5/16 -> Delay91/1, CMult91/1  "<signal16>"
  Bus Selector5/3 -> Delay97/1, CMult97/1  "<signal3>"
  AddSub97/1 -> AddSub100/2
  Bus Selector5/8 -> Delay83/1, CMult83/1  "<signal8>"
  CMult87/1 -> AddSub103/1
  CMult89/1 -> AddSub104/1
  Bus Selector5/1 -> Delay79/1, CMult79/1  "<signal1>"
  Bus Selector5/6 -> Delay81/1, CMult81/1  "<signal6>"
  CMult96/1 -> AddSub111/1
  Bus Selector5/18 -> CMult92/1, Delay92/1  "<signal18>"
  CMult84/1 -> AddSub99/1
  Bus Selector5/4 -> Delay80/1, CMult80/1  "<signal4>"
  AddSub102/1 -> AddSub104/2
  Delay85/1 -> Bus Creator6/9
  CMult81/1 -> AddSub96/1
  AddSub112/1 -> AddSub95/2
  Delay80/1 -> Bus Creator6/4
  AddSub109/1 -> AddSub107/2
  Delay96/1 -> Bus Creator6/19
  Bus Selector5/5 -> Delay82/1, CMult82/1  "<signal5>"
  CMult79/1 -> AddSub103/2
  CMult90/1 -> AddSub102/1
  AddSub105/1 -> AddSub109/2
  CMult83/1 -> AddSub100/1
  AddSub95/1 -> AddSub96/2
  Bus Selector5/11 -> Delay95/1, CMult95/1  "<signal11>"
  CMult101/1 -> AddSub114/1
  Delay111/1 -> Bus Creator7/16
  Delay107/1 -> Bus Creator7/2
  AddSub123/1 -> AddSub124/2
  AddSub126/1 -> AddSub129/2
  CMult114/1 -> AddSub124/1
  Bus Selector6/7 -> Delay106/1, CMult105/1  "<signal7>"
  Bus Creator6/1 -> Bus Selector6/1
  AddSub115/1 -> AddSub116/2
  Delay114/1 -> Bus Creator7/15
  CMult104/1 -> AddSub117/1
  AddSub113/1 -> AddSub130/2
  Delay106/1 -> Bus Creator7/7
  Delay102/1 -> Bus Creator7/8
  CMult113/1 -> AddSub125/1
  AddSub120/1 -> AddSub128/2
  Delay117/1 -> Bus Creator7/3
  Bus Selector6/2 -> Delay107/1, CMult106/1  "<signal2>"
  CMult112/1 -> AddSub126/1
  Delay98/1 -> Bus Creator7/1
  CMult117/1 -> AddSub113/1
  Bus Selector6/19 -> CMult116/1, Delay116/1  "<signal19>"
  Delay101/1 -> Bus Creator7/5
  AddSub122/1 -> AddSub113/2
  AddSub125/1 -> AddSub126/2
  Bus Selector6/13 -> Delay110/1, CMult109/1  "<signal13>"
  Bus Selector6/10 -> CMult103/1, Delay103/1  "<signal10>"
  CMult115/1 -> AddSub120/1
  AddSub118/1 -> AddSub120/2
  CMult107/1 -> AddSub128/1
  CMult105/1 -> AddSub116/1
  Delay108/1 -> Bus Creator7/12
  Delay109/1 -> Bus Creator7/14
  Bus Selector6/12 -> Delay108/1, CMult107/1  "<signal12>"
  CMult111/1 -> AddSub127/1
  Delay112/1 -> Bus Creator7/18
  Bus Selector6/15 -> Delay114/1, CMult114/1  "<signal15>"
  Bus Selector6/9 -> Delay105/1, CMult104/1  "<signal9>"
  AddSub128/1 -> AddSub121/2
  Delay110/1 -> Bus Creator7/13
  Delay103/1 -> Bus Creator7/10
  Bus Selector6/17 -> Delay113/1, CMult113/1  "<signal17>"
  Delay100/1 -> Bus Creator7/6
  AddSub119/1 -> AddSub117/2
  Delay113/1 -> Bus Creator7/17
  Delay115/1 -> Bus Creator7/11
  Bus Selector6/14 -> Delay109/1, CMult108/1  "<signal14>"
  CMult99/1 -> AddSub130/1
  AddSub117/1 -> AddSub118/2
  Bus Selector6/16 -> Delay111/1, CMult111/1  "<signal16>"
  Bus Selector6/3 -> Delay117/1, CMult117/1  "<signal3>"
  AddSub116/1 -> AddSub119/2
  Bus Selector6/8 -> Delay102/1, CMult102/1  "<signal8>"
  CMult106/1 -> AddSub122/1
  CMult108/1 -> AddSub123/1
  Bus Selector6/1 -> Delay98/1, CMult98/1  "<signal1>"
  Bus Selector6/6 -> Delay100/1, CMult100/1  "<signal6>"
  CMult116/1 -> AddSub129/1
  Bus Selector6/18 -> CMult112/1, Delay112/1  "<signal18>"
  CMult103/1 -> AddSub118/1
  Bus Selector6/4 -> Delay99/1, CMult99/1  "<signal4>"
  AddSub121/1 -> AddSub123/2
  Delay105/1 -> Bus Creator7/9
  CMult100/1 -> AddSub115/1
  AddSub130/1 -> AddSub114/2
  Delay99/1 -> Bus Creator7/4
  AddSub127/1 -> AddSub125/2
  Delay116/1 -> Bus Creator7/19
  Bus Selector6/5 -> Delay101/1, CMult101/1  "<signal5>"
  CMult98/1 -> AddSub122/2
  CMult109/1 -> AddSub121/1
  AddSub124/1 -> AddSub127/2
  CMult102/1 -> AddSub119/1
  AddSub114/1 -> AddSub115/2
  Bus Selector6/11 -> Delay115/1, CMult115/1  "<signal11>"
  CMult121/1 -> AddSub132/1
  Delay130/1 -> Bus Creator8/16
  Delay126/1 -> Bus Creator8/2
  AddSub141/1 -> AddSub142/2
  AddSub144/1 -> AddSub148/2
  CMult133/1 -> AddSub142/1
  Bus Selector7/7 -> Delay125/1, CMult125/1  "<signal7>"
  Bus Creator7/1 -> Bus Selector7/1
  AddSub133/1 -> AddSub134/2
  Delay133/1 -> Bus Creator8/15
  CMult124/1 -> AddSub135/1
  AddSub131/1 -> AddSub149/2
  Delay125/1 -> Bus Creator8/7
  Delay122/1 -> Bus Creator8/8
  CMult132/1 -> AddSub143/1
  AddSub138/1 -> AddSub147/2
  Delay136/1 -> Bus Creator8/3
  Bus Selector7/2 -> Delay126/1, CMult126/1  "<signal2>"
  CMult131/1 -> AddSub144/1
  Delay118/1 -> Bus Creator8/1
  CMult136/1 -> AddSub131/1
  Bus Selector7/19 -> CMult135/1, Delay135/1  "<signal19>"
  Delay121/1 -> Bus Creator8/5
  AddSub140/1 -> AddSub131/2
  AddSub143/1 -> AddSub144/2
  Bus Selector7/13 -> Delay129/1, CMult129/1  "<signal13>"
  Bus Selector7/10 -> CMult123/1, Delay123/1  "<signal10>"
  CMult134/1 -> AddSub138/1
  AddSub136/1 -> AddSub138/2
  CMult127/1 -> AddSub147/1
  CMult125/1 -> AddSub134/1
  Delay127/1 -> Bus Creator8/12
  Delay128/1 -> Bus Creator8/14
  Bus Selector7/12 -> Delay127/1, CMult127/1  "<signal12>"
  CMult130/1 -> AddSub146/1
  Delay131/1 -> Bus Creator8/18
  Bus Selector7/15 -> Delay133/1, CMult133/1  "<signal15>"
  Bus Selector7/9 -> Delay124/1, CMult124/1  "<signal9>"
  AddSub147/1 -> AddSub139/2
  Delay129/1 -> Bus Creator8/13
  Delay123/1 -> Bus Creator8/10
  Bus Selector7/17 -> Delay132/1, CMult132/1  "<signal17>"
  Delay120/1 -> Bus Creator8/6
  AddSub137/1 -> AddSub135/2
  Delay132/1 -> Bus Creator8/17
  Delay134/1 -> Bus Creator8/11
  Bus Selector7/14 -> Delay128/1, CMult128/1  "<signal14>"
  CMult119/1 -> AddSub149/1
  AddSub135/1 -> AddSub136/2
  Bus Selector7/16 -> Delay130/1, CMult130/1  "<signal16>"
  Bus Selector7/3 -> Delay136/1, CMult136/1  "<signal3>"
  AddSub134/1 -> AddSub137/2
  Bus Selector7/8 -> Delay122/1, CMult122/1  "<signal8>"
  CMult126/1 -> AddSub140/1
  CMult128/1 -> AddSub141/1
  Bus Selector7/1 -> Delay118/1, CMult118/1  "<signal1>"
  Bus Selector7/6 -> Delay120/1, CMult120/1  "<signal6>"
  CMult135/1 -> AddSub148/1
  Bus Selector7/18 -> CMult131/1, Delay131/1  "<signal18>"
  CMult123/1 -> AddSub136/1
  Bus Selector7/4 -> Delay119/1, CMult119/1  "<signal4>"
  AddSub139/1 -> AddSub141/2
  Delay124/1 -> Bus Creator8/9
  CMult120/1 -> AddSub133/1
  AddSub149/1 -> AddSub132/2
  Delay119/1 -> Bus Creator8/4
  AddSub146/1 -> AddSub143/2
  Delay135/1 -> Bus Creator8/19
  Bus Selector7/5 -> Delay121/1, CMult121/1  "<signal5>"
  CMult118/1 -> AddSub140/2
  CMult129/1 -> AddSub139/1
  AddSub142/1 -> AddSub146/2
  CMult122/1 -> AddSub137/1
  AddSub132/1 -> AddSub133/2
  Bus Selector7/11 -> Delay134/1, CMult134/1  "<signal11>"
  CMult140/1 -> AddSub151/1
  Delay150/1 -> Bus Creator9/16
  Delay146/1 -> Bus Creator9/2
  AddSub160/1 -> AddSub161/2
  AddSub163/1 -> AddSub166/2
  CMult153/1 -> AddSub161/1
  Bus Selector8/7 -> Delay145/1, CMult144/1  "<signal7>"
  Bus Creator8/1 -> Bus Selector8/1
  AddSub152/1 -> AddSub153/2
  Delay153/1 -> Bus Creator9/15
  CMult143/1 -> AddSub154/1
  AddSub150/1 -> AddSub167/2
  Delay145/1 -> Bus Creator9/7
  Delay142/1 -> Bus Creator9/8
  CMult152/1 -> AddSub162/1
  AddSub157/1 -> AddSub165/2
  Delay156/1 -> Bus Creator9/3
  Bus Selector8/2 -> Delay146/1, CMult145/1  "<signal2>"
  CMult151/1 -> AddSub163/1
  Delay137/1 -> Bus Creator9/1
  CMult156/1 -> AddSub150/1
  Bus Selector8/19 -> CMult155/1, Delay155/1  "<signal19>"
  Delay141/1 -> Bus Creator9/5
  AddSub159/1 -> AddSub150/2
  AddSub162/1 -> AddSub163/2
  Bus Selector8/13 -> Delay149/1, CMult148/1  "<signal13>"
  Bus Selector8/10 -> CMult142/1, Delay143/1  "<signal10>"
  CMult154/1 -> AddSub157/1
  AddSub155/1 -> AddSub157/2
  CMult146/1 -> AddSub165/1
  CMult144/1 -> AddSub153/1
  Delay147/1 -> Bus Creator9/12
  Delay148/1 -> Bus Creator9/14
  Bus Selector8/12 -> Delay147/1, CMult146/1  "<signal12>"
  CMult149/1 -> AddSub164/1
  Delay151/1 -> Bus Creator9/18
  Bus Selector8/15 -> Delay153/1, CMult153/1  "<signal15>"
  Bus Selector8/9 -> Delay144/1, CMult143/1  "<signal9>"
  AddSub165/1 -> AddSub158/2
  Delay149/1 -> Bus Creator9/13
  Delay143/1 -> Bus Creator9/10
  Bus Selector8/17 -> Delay152/1, CMult152/1  "<signal17>"
  Delay139/1 -> Bus Creator9/6
  AddSub156/1 -> AddSub154/2
  Delay152/1 -> Bus Creator9/17
  Delay154/1 -> Bus Creator9/11
  Bus Selector8/14 -> Delay148/1, CMult147/1  "<signal14>"
  CMult138/1 -> AddSub167/1
  AddSub154/1 -> AddSub155/2
  Bus Selector8/16 -> Delay150/1, CMult149/1  "<signal16>"
  Bus Selector8/3 -> Delay156/1, CMult156/1  "<signal3>"
  AddSub153/1 -> AddSub156/2
  Bus Selector8/8 -> Delay142/1, CMult141/1  "<signal8>"
  CMult145/1 -> AddSub159/1
  CMult147/1 -> AddSub160/1
  Bus Selector8/1 -> Delay137/1, CMult137/1  "<signal1>"
  Bus Selector8/6 -> Delay139/1, CMult139/1  "<signal6>"
  CMult155/1 -> AddSub166/1
  Bus Selector8/18 -> CMult151/1, Delay151/1  "<signal18>"
  CMult142/1 -> AddSub155/1
  Bus Selector8/4 -> Delay138/1, CMult138/1  "<signal4>"
  AddSub158/1 -> AddSub160/2
  Delay144/1 -> Bus Creator9/9
  CMult139/1 -> AddSub152/1
  AddSub167/1 -> AddSub151/2
  Delay138/1 -> Bus Creator9/4
  AddSub164/1 -> AddSub162/2
  Delay155/1 -> Bus Creator9/19
  Bus Selector8/5 -> Delay141/1, CMult140/1  "<signal5>"
  CMult137/1 -> AddSub159/2
  CMult148/1 -> AddSub158/1
  AddSub161/1 -> AddSub164/2
  CMult141/1 -> AddSub156/1
  AddSub151/1 -> AddSub152/2
  Bus Selector8/11 -> Delay154/1, CMult154/1  "<signal11>"
  CMult160/1 -> AddSub169/1
  Delay169/1 -> Bus Creator10/16
  Delay165/1 -> Bus Creator10/2
  AddSub179/1 -> AddSub180/2
  AddSub182/1 -> AddSub186/2
  CMult172/1 -> AddSub180/1
  Bus Selector9/7 -> Delay164/1, CMult164/1  "<signal7>"
  Bus Creator9/1 -> Bus Selector9/1
  AddSub170/1 -> AddSub171/2
  Delay173/1 -> Bus Creator10/15
  CMult163/1 -> AddSub172/1
  AddSub168/1 -> AddSub187/2
  Delay164/1 -> Bus Creator10/7
  Delay161/1 -> Bus Creator10/8
  CMult171/1 -> AddSub181/1
  AddSub175/1 -> AddSub185/2
  Delay176/1 -> Bus Creator10/3
  Bus Selector9/2 -> Delay165/1, CMult165/1  "<signal2>"
  CMult170/1 -> AddSub182/1
  Delay157/1 -> Bus Creator10/1
  CMult175/1 -> AddSub168/1
  Bus Selector9/19 -> CMult174/1, Delay175/1  "<signal19>"
  Delay160/1 -> Bus Creator10/5
  AddSub178/1 -> AddSub168/2
  AddSub181/1 -> AddSub182/2
  Bus Selector9/13 -> Delay168/1, CMult168/1  "<signal13>"
  Bus Selector9/10 -> CMult162/1, Delay162/1  "<signal10>"
  CMult173/1 -> AddSub175/1
  AddSub173/1 -> AddSub175/2
  CMult166/1 -> AddSub185/1
  CMult164/1 -> AddSub171/1
  Delay166/1 -> Bus Creator10/12
  Delay167/1 -> Bus Creator10/14
  Bus Selector9/12 -> Delay166/1, CMult166/1  "<signal12>"
  CMult169/1 -> AddSub183/1
  Delay170/1 -> Bus Creator10/18
  Bus Selector9/15 -> Delay173/1, CMult172/1  "<signal15>"
  Bus Selector9/9 -> Delay163/1, CMult163/1  "<signal9>"
  AddSub185/1 -> AddSub177/2
  Delay168/1 -> Bus Creator10/13
  Delay162/1 -> Bus Creator10/10
  Bus Selector9/17 -> Delay171/1, CMult171/1  "<signal17>"
  Delay159/1 -> Bus Creator10/6
  AddSub174/1 -> AddSub172/2
  Delay171/1 -> Bus Creator10/17
  Delay174/1 -> Bus Creator10/11
  Bus Selector9/14 -> Delay167/1, CMult167/1  "<signal14>"
  CMult158/1 -> AddSub187/1
  AddSub172/1 -> AddSub173/2
  Bus Selector9/16 -> Delay169/1, CMult169/1  "<signal16>"
  Bus Selector9/3 -> Delay176/1, CMult175/1  "<signal3>"
  AddSub171/1 -> AddSub174/2
  Bus Selector9/8 -> Delay161/1, CMult161/1  "<signal8>"
  CMult165/1 -> AddSub178/1
  CMult167/1 -> AddSub179/1
  Bus Selector9/1 -> Delay157/1, CMult157/1  "<signal1>"
  Bus Selector9/6 -> Delay159/1, CMult159/1  "<signal6>"
  CMult174/1 -> AddSub186/1
  Bus Selector9/18 -> CMult170/1, Delay170/1  "<signal18>"
  CMult162/1 -> AddSub173/1
  Bus Selector9/4 -> Delay158/1, CMult158/1  "<signal4>"
  AddSub177/1 -> AddSub179/2
  Delay163/1 -> Bus Creator10/9
  CMult159/1 -> AddSub170/1
  AddSub187/1 -> AddSub169/2
  Delay158/1 -> Bus Creator10/4
  AddSub183/1 -> AddSub181/2
  Delay175/1 -> Bus Creator10/19
  Bus Selector9/5 -> Delay160/1, CMult160/1  "<signal5>"
  CMult157/1 -> AddSub178/2
  CMult168/1 -> AddSub177/1
  AddSub180/1 -> AddSub183/2
  CMult161/1 -> AddSub174/1
  AddSub169/1 -> AddSub170/2
  Bus Selector9/11 -> Delay174/1, CMult173/1  "<signal11>"
  CMult179/1 -> AddSub189/1
  Delay189/1 -> Bus Creator11/16
  Delay185/1 -> Bus Creator11/2
  AddSub198/1 -> AddSub199/2
  AddSub201/1 -> AddSub204/2
  CMult192/1 -> AddSub199/1
  Bus Selector10/7 -> Delay184/1, CMult184/1  "<signal7>"
  Bus Creator10/1 -> Bus Selector10/1
  AddSub190/1 -> AddSub191/2
  Delay192/1 -> Bus Creator11/15
  CMult183/1 -> AddSub192/1
  AddSub188/1 -> AddSub205/2
  Delay184/1 -> Bus Creator11/7
  Delay181/1 -> Bus Creator11/8
  CMult191/1 -> AddSub200/1
  AddSub195/1 -> AddSub203/2
  Delay195/1 -> Bus Creator11/3
  Bus Selector10/2 -> Delay185/1, CMult185/1  "<signal2>"
  CMult190/1 -> AddSub201/1
  Delay177/1 -> Bus Creator11/1
  CMult195/1 -> AddSub188/1
  Bus Selector10/19 -> CMult194/1, Delay194/1  "<signal19>"
  Delay180/1 -> Bus Creator11/5
  AddSub197/1 -> AddSub188/2
  AddSub200/1 -> AddSub201/2
  Bus Selector10/13 -> Delay188/1, CMult188/1  "<signal13>"
  Bus Selector10/10 -> CMult182/1, Delay182/1  "<signal10>"
  CMult193/1 -> AddSub195/1
  AddSub193/1 -> AddSub195/2
  CMult186/1 -> AddSub203/1
  CMult184/1 -> AddSub191/1
  Delay186/1 -> Bus Creator11/12
  Delay187/1 -> Bus Creator11/14
  Bus Selector10/12 -> Delay186/1, CMult186/1  "<signal12>"
  CMult189/1 -> AddSub202/1
  Delay190/1 -> Bus Creator11/18
  Bus Selector10/15 -> Delay192/1, CMult192/1  "<signal15>"
  Bus Selector10/9 -> Delay183/1, CMult183/1  "<signal9>"
  AddSub203/1 -> AddSub196/2
  Delay188/1 -> Bus Creator11/13
  Delay182/1 -> Bus Creator11/10
  Bus Selector10/17 -> Delay191/1, CMult191/1  "<signal17>"
  Delay179/1 -> Bus Creator11/6
  AddSub194/1 -> AddSub192/2
  Delay191/1 -> Bus Creator11/17
  Delay193/1 -> Bus Creator11/11
  Bus Selector10/14 -> Delay187/1, CMult187/1  "<signal14>"
  CMult177/1 -> AddSub205/1
  AddSub192/1 -> AddSub193/2
  Bus Selector10/16 -> Delay189/1, CMult189/1  "<signal16>"
  Bus Selector10/3 -> Delay195/1, CMult195/1  "<signal3>"
  AddSub191/1 -> AddSub194/2
  Bus Selector10/8 -> Delay181/1, CMult181/1  "<signal8>"
  CMult185/1 -> AddSub197/1
  CMult187/1 -> AddSub198/1
  Bus Selector10/1 -> Delay177/1, CMult176/1  "<signal1>"
  Bus Selector10/6 -> Delay179/1, CMult178/1  "<signal6>"
  CMult194/1 -> AddSub204/1
  Bus Selector10/18 -> CMult190/1, Delay190/1  "<signal18>"
  CMult182/1 -> AddSub193/1
  Bus Selector10/4 -> Delay178/1, CMult177/1  "<signal4>"
  AddSub196/1 -> AddSub198/2
  Delay183/1 -> Bus Creator11/9
  CMult178/1 -> AddSub190/1
  AddSub205/1 -> AddSub189/2
  Delay178/1 -> Bus Creator11/4
  AddSub202/1 -> AddSub200/2
  Delay194/1 -> Bus Creator11/19
  Bus Selector10/5 -> Delay180/1, CMult179/1  "<signal5>"
  CMult176/1 -> AddSub197/2
  CMult188/1 -> AddSub196/1
  AddSub199/1 -> AddSub202/2
  CMult181/1 -> AddSub194/1
  AddSub189/1 -> AddSub190/2
  Bus Selector10/11 -> Delay193/1, CMult193/1  "<signal11>"
  CMult199/1 -> AddSub207/1
  Delay209/1 -> Bus Creator12/16
  Delay204/1 -> Bus Creator12/2
  AddSub216/1 -> AddSub217/2
  AddSub219/1 -> AddSub222/2
  CMult211/1 -> AddSub217/1
  Bus Selector11/7 -> Delay203/1, CMult203/1  "<signal7>"
  Bus Creator11/1 -> Bus Selector11/1
  AddSub208/1 -> AddSub209/2
  Delay212/1 -> Bus Creator12/15
  CMult202/1 -> AddSub210/1
  AddSub206/1 -> AddSub223/2
  Delay203/1 -> Bus Creator12/7
  Delay200/1 -> Bus Creator12/8
  CMult210/1 -> AddSub218/1
  AddSub213/1 -> AddSub221/2
  Delay215/1 -> Bus Creator12/3
  Bus Selector11/2 -> Delay204/1, CMult204/1  "<signal2>"
  CMult209/1 -> AddSub219/1
  Delay196/1 -> Bus Creator12/1
  CMult214/1 -> AddSub206/1
  Bus Selector11/19 -> CMult213/1, Delay214/1  "<signal19>"
  Delay199/1 -> Bus Creator12/5
  AddSub215/1 -> AddSub206/2
  AddSub218/1 -> AddSub219/2
  Bus Selector11/13 -> Delay207/1, CMult207/1  "<signal13>"
  Bus Selector11/10 -> CMult201/1, Delay201/1  "<signal10>"
  CMult212/1 -> AddSub213/1
  AddSub211/1 -> AddSub213/2
  CMult205/1 -> AddSub221/1
  CMult203/1 -> AddSub209/1
  Delay205/1 -> Bus Creator12/12
  Delay206/1 -> Bus Creator12/14
  Bus Selector11/12 -> Delay205/1, CMult205/1  "<signal12>"
  CMult208/1 -> AddSub220/1
  Delay210/1 -> Bus Creator12/18
  Bus Selector11/15 -> Delay212/1, CMult211/1  "<signal15>"
  Bus Selector11/9 -> Delay202/1, CMult202/1  "<signal9>"
  AddSub221/1 -> AddSub214/2
  Delay207/1 -> Bus Creator12/13
  Delay201/1 -> Bus Creator12/10
  Bus Selector11/17 -> Delay211/1, CMult210/1  "<signal17>"
  Delay198/1 -> Bus Creator12/6
  AddSub212/1 -> AddSub210/2
  Delay211/1 -> Bus Creator12/17
  Delay213/1 -> Bus Creator12/11
  Bus Selector11/14 -> Delay206/1, CMult206/1  "<signal14>"
  CMult197/1 -> AddSub223/1
  AddSub210/1 -> AddSub211/2
  Bus Selector11/16 -> Delay209/1, CMult208/1  "<signal16>"
  Bus Selector11/3 -> Delay215/1, CMult214/1  "<signal3>"
  AddSub209/1 -> AddSub212/2
  Bus Selector11/8 -> Delay200/1, CMult200/1  "<signal8>"
  CMult204/1 -> AddSub215/1
  CMult206/1 -> AddSub216/1
  Bus Selector11/1 -> Delay196/1, CMult196/1  "<signal1>"
  Bus Selector11/6 -> Delay198/1, CMult198/1  "<signal6>"
  CMult213/1 -> AddSub222/1
  Bus Selector11/18 -> CMult209/1, Delay210/1  "<signal18>"
  CMult201/1 -> AddSub211/1
  Bus Selector11/4 -> Delay197/1, CMult197/1  "<signal4>"
  AddSub214/1 -> AddSub216/2
  Delay202/1 -> Bus Creator12/9
  CMult198/1 -> AddSub208/1
  AddSub223/1 -> AddSub207/2
  Delay197/1 -> Bus Creator12/4
  AddSub220/1 -> AddSub218/2
  Delay214/1 -> Bus Creator12/19
  Bus Selector11/5 -> Delay199/1, CMult199/1  "<signal5>"
  CMult196/1 -> AddSub215/2
  CMult207/1 -> AddSub214/1
  AddSub217/1 -> AddSub220/2
  CMult200/1 -> AddSub212/1
  AddSub207/1 -> AddSub208/2
  Bus Selector11/11 -> Delay213/1, CMult212/1  "<signal11>"
  CMult218/1 -> AddSub225/1
  Delay228/1 -> Bus Creator13/16
  Delay224/1 -> Bus Creator13/2
  AddSub235/1 -> AddSub236/2
  AddSub238/1 -> AddSub241/2
  CMult231/1 -> AddSub236/1
  Bus Selector12/7 -> Delay223/1, CMult223/1  "<signal7>"
  Bus Creator12/1 -> Bus Selector12/1
  AddSub226/1 -> AddSub228/2
  Delay231/1 -> Bus Creator13/15
  CMult222/1 -> AddSub229/1
  AddSub224/1 -> AddSub242/2
  Delay223/1 -> Bus Creator13/7
  Delay220/1 -> Bus Creator13/8
  CMult230/1 -> AddSub237/1
  AddSub232/1 -> AddSub240/2
  Delay234/1 -> Bus Creator13/3
  Bus Selector12/2 -> Delay224/1, CMult224/1  "<signal2>"
  CMult229/1 -> AddSub238/1
  Delay216/1 -> Bus Creator13/1
  CMult234/1 -> AddSub224/1
  Bus Selector12/19 -> CMult233/1, Delay233/1  "<signal19>"
  Delay219/1 -> Bus Creator13/5
  AddSub234/1 -> AddSub224/2
  AddSub237/1 -> AddSub238/2
  Bus Selector12/13 -> Delay227/1, CMult227/1  "<signal13>"
  Bus Selector12/10 -> CMult221/1, Delay221/1  "<signal10>"
  CMult232/1 -> AddSub232/1
  AddSub230/1 -> AddSub232/2
  CMult225/1 -> AddSub240/1
  CMult223/1 -> AddSub228/1
  Delay225/1 -> Bus Creator13/12
  Delay226/1 -> Bus Creator13/14
  Bus Selector12/12 -> Delay225/1, CMult225/1  "<signal12>"
  CMult228/1 -> AddSub239/1
  Delay229/1 -> Bus Creator13/18
  Bus Selector12/15 -> Delay231/1, CMult231/1  "<signal15>"
  Bus Selector12/9 -> Delay222/1, CMult222/1  "<signal9>"
  AddSub240/1 -> AddSub233/2
  Delay227/1 -> Bus Creator13/13
  Delay221/1 -> Bus Creator13/10
  Bus Selector12/17 -> Delay230/1, CMult230/1  "<signal17>"
  Delay218/1 -> Bus Creator13/6
  AddSub231/1 -> AddSub229/2
  Delay230/1 -> Bus Creator13/17
  Delay232/1 -> Bus Creator13/11
  Bus Selector12/14 -> Delay226/1, CMult226/1  "<signal14>"
  CMult216/1 -> AddSub242/1
  AddSub229/1 -> AddSub230/2
  Bus Selector12/16 -> Delay228/1, CMult228/1  "<signal16>"
  Bus Selector12/3 -> Delay234/1, CMult234/1  "<signal3>"
  AddSub228/1 -> AddSub231/2
  Bus Selector12/8 -> Delay220/1, CMult219/1  "<signal8>"
  CMult224/1 -> AddSub234/1
  CMult226/1 -> AddSub235/1
  Bus Selector12/1 -> Delay216/1, CMult215/1  "<signal1>"
  Bus Selector12/6 -> Delay218/1, CMult217/1  "<signal6>"
  CMult233/1 -> AddSub241/1
  Bus Selector12/18 -> CMult229/1, Delay229/1  "<signal18>"
  CMult221/1 -> AddSub230/1
  Bus Selector12/4 -> Delay217/1, CMult216/1  "<signal4>"
  AddSub233/1 -> AddSub235/2
  Delay222/1 -> Bus Creator13/9
  CMult217/1 -> AddSub226/1
  AddSub242/1 -> AddSub225/2
  Delay217/1 -> Bus Creator13/4
  AddSub239/1 -> AddSub237/2
  Delay233/1 -> Bus Creator13/19
  Bus Selector12/5 -> Delay219/1, CMult218/1  "<signal5>"
  CMult215/1 -> AddSub234/2
  CMult227/1 -> AddSub233/1
  AddSub236/1 -> AddSub239/2
  CMult219/1 -> AddSub231/1
  AddSub225/1 -> AddSub226/2
  Bus Selector12/11 -> Delay232/1, CMult232/1  "<signal11>"
  CMult238/1 -> AddSub244/1
  Delay248/1 -> Bus Creator14/16
  Delay243/1 -> Bus Creator14/2
  AddSub253/1 -> AddSub254/2
  AddSub256/1 -> AddSub259/2
  CMult250/1 -> AddSub254/1
  Bus Selector13/7 -> Delay242/1, CMult242/1  "<signal7>"
  Bus Creator13/1 -> Bus Selector13/1
  AddSub245/1 -> AddSub246/2
  Delay251/1 -> Bus Creator14/15
  CMult241/1 -> AddSub247/1
  AddSub243/1 -> AddSub260/2
  Delay242/1 -> Bus Creator14/7
  Delay239/1 -> Bus Creator14/8
  CMult249/1 -> AddSub255/1
  AddSub250/1 -> AddSub258/2
  Delay254/1 -> Bus Creator14/3
  Bus Selector13/2 -> Delay243/1, CMult243/1  "<signal2>"
  CMult248/1 -> AddSub256/1
  Delay235/1 -> Bus Creator14/1
  CMult253/1 -> AddSub243/1
  Bus Selector13/19 -> CMult252/1, Delay253/1  "<signal19>"
  Delay238/1 -> Bus Creator14/5
  AddSub252/1 -> AddSub243/2
  AddSub255/1 -> AddSub256/2
  Bus Selector13/13 -> Delay247/1, CMult246/1  "<signal13>"
  Bus Selector13/10 -> CMult240/1, Delay240/1  "<signal10>"
  CMult251/1 -> AddSub250/1
  AddSub248/1 -> AddSub250/2
  CMult244/1 -> AddSub258/1
  CMult242/1 -> AddSub246/1
  Delay245/1 -> Bus Creator14/12
  Delay246/1 -> Bus Creator14/14
  Bus Selector13/12 -> Delay245/1, CMult244/1  "<signal12>"
  CMult247/1 -> AddSub257/1
  Delay249/1 -> Bus Creator14/18
  Bus Selector13/15 -> Delay251/1, CMult250/1  "<signal15>"
  Bus Selector13/9 -> Delay241/1, CMult241/1  "<signal9>"
  AddSub258/1 -> AddSub251/2
  Delay247/1 -> Bus Creator14/13
  Delay240/1 -> Bus Creator14/10
  Bus Selector13/17 -> Delay250/1, CMult249/1  "<signal17>"
  Delay237/1 -> Bus Creator14/6
  AddSub249/1 -> AddSub247/2
  Delay250/1 -> Bus Creator14/17
  Delay252/1 -> Bus Creator14/11
  Bus Selector13/14 -> Delay246/1, CMult245/1  "<signal14>"
  CMult236/1 -> AddSub260/1
  AddSub247/1 -> AddSub248/2
  Bus Selector13/16 -> Delay248/1, CMult247/1  "<signal16>"
  Bus Selector13/3 -> Delay254/1, CMult253/1  "<signal3>"
  AddSub246/1 -> AddSub249/2
  Bus Selector13/8 -> Delay239/1, CMult239/1  "<signal8>"
  CMult243/1 -> AddSub252/1
  CMult245/1 -> AddSub253/1
  Bus Selector13/1 -> Delay235/1, CMult235/1  "<signal1>"
  Bus Selector13/6 -> Delay237/1, CMult237/1  "<signal6>"
  CMult252/1 -> AddSub259/1
  Bus Selector13/18 -> CMult248/1, Delay249/1  "<signal18>"
  CMult240/1 -> AddSub248/1
  Bus Selector13/4 -> Delay236/1, CMult236/1  "<signal4>"
  AddSub251/1 -> AddSub253/2
  Delay241/1 -> Bus Creator14/9
  CMult237/1 -> AddSub245/1
  AddSub260/1 -> AddSub244/2
  Delay236/1 -> Bus Creator14/4
  AddSub257/1 -> AddSub255/2
  Delay253/1 -> Bus Creator14/19
  Bus Selector13/5 -> Delay238/1, CMult238/1  "<signal5>"
  CMult235/1 -> AddSub252/2
  CMult246/1 -> AddSub251/1
  AddSub254/1 -> AddSub257/2
  CMult239/1 -> AddSub249/1
  AddSub244/1 -> AddSub245/2
  Bus Selector13/11 -> Delay252/1, CMult251/1  "<signal11>"
  CMult257/1 -> AddSub262/1
  Delay267/1 -> Bus Creator15/16
  Delay263/1 -> Bus Creator15/2
  AddSub271/1 -> AddSub272/2
  AddSub274/1 -> AddSub277/2
  CMult270/1 -> AddSub272/1
  Bus Selector14/7 -> Delay262/1, CMult262/1  "<signal7>"
  Bus Creator14/1 -> Bus Selector14/1
  AddSub263/1 -> AddSub264/2
  Delay270/1 -> Bus Creator15/15
  CMult261/1 -> AddSub265/1
  AddSub261/1 -> AddSub278/2
  Delay262/1 -> Bus Creator15/7
  Delay259/1 -> Bus Creator15/8
  CMult269/1 -> AddSub273/1
  AddSub268/1 -> AddSub276/2
  Delay273/1 -> Bus Creator15/3
  Bus Selector14/2 -> Delay263/1, CMult263/1  "<signal2>"
  CMult268/1 -> AddSub274/1
  Delay255/1 -> Bus Creator15/1
  CMult273/1 -> AddSub261/1
  Bus Selector14/19 -> CMult272/1, Delay272/1  "<signal19>"
  Delay258/1 -> Bus Creator15/5
  AddSub270/1 -> AddSub261/2
  AddSub273/1 -> AddSub274/2
  Bus Selector14/13 -> Delay266/1, CMult266/1  "<signal13>"
  Bus Selector14/10 -> CMult259/1, Delay260/1  "<signal10>"
  CMult271/1 -> AddSub268/1
  AddSub266/1 -> AddSub268/2
  CMult264/1 -> AddSub276/1
  CMult262/1 -> AddSub264/1
  Delay264/1 -> Bus Creator15/12
  Delay265/1 -> Bus Creator15/14
  Bus Selector14/12 -> Delay264/1, CMult264/1  "<signal12>"
  CMult267/1 -> AddSub275/1
  Delay268/1 -> Bus Creator15/18
  Bus Selector14/15 -> Delay270/1, CMult270/1  "<signal15>"
  Bus Selector14/9 -> Delay261/1, CMult261/1  "<signal9>"
  AddSub276/1 -> AddSub269/2
  Delay266/1 -> Bus Creator15/13
  Delay260/1 -> Bus Creator15/10
  Bus Selector14/17 -> Delay269/1, CMult269/1  "<signal17>"
  Delay257/1 -> Bus Creator15/6
  AddSub267/1 -> AddSub265/2
  Delay269/1 -> Bus Creator15/17
  Delay271/1 -> Bus Creator15/11
  Bus Selector14/14 -> Delay265/1, CMult265/1  "<signal14>"
  CMult255/1 -> AddSub278/1
  AddSub265/1 -> AddSub266/2
  Bus Selector14/16 -> Delay267/1, CMult267/1  "<signal16>"
  Bus Selector14/3 -> Delay273/1, CMult273/1  "<signal3>"
  AddSub264/1 -> AddSub267/2
  Bus Selector14/8 -> Delay259/1, CMult258/1  "<signal8>"
  CMult263/1 -> AddSub270/1
  CMult265/1 -> AddSub271/1
  Bus Selector14/1 -> Delay255/1, CMult254/1  "<signal1>"
  Bus Selector14/6 -> Delay257/1, CMult256/1  "<signal6>"
  CMult272/1 -> AddSub277/1
  Bus Selector14/18 -> CMult268/1, Delay268/1  "<signal18>"
  CMult259/1 -> AddSub266/1
  Bus Selector14/4 -> Delay256/1, CMult255/1  "<signal4>"
  AddSub269/1 -> AddSub271/2
  Delay261/1 -> Bus Creator15/9
  CMult256/1 -> AddSub263/1
  AddSub278/1 -> AddSub262/2
  Delay256/1 -> Bus Creator15/4
  AddSub275/1 -> AddSub273/2
  Delay272/1 -> Bus Creator15/19
  Bus Selector14/5 -> Delay258/1, CMult257/1  "<signal5>"
  CMult254/1 -> AddSub270/2
  CMult266/1 -> AddSub269/1
  AddSub272/1 -> AddSub275/2
  CMult258/1 -> AddSub267/1
  AddSub262/1 -> AddSub263/2
  Bus Selector14/11 -> Delay271/1, CMult271/1  "<signal11>"
  CMult277/1 -> AddSub280/1
  Delay287/1 -> Bus Creator16/16
  Delay283/1 -> Bus Creator16/2
  AddSub290/1 -> AddSub291/2
  AddSub293/1 -> AddSub296/2
  CMult289/1 -> AddSub291/1
  Bus Selector15/7 -> Delay282/1, CMult281/1  "<signal7>"
  Bus Creator15/1 -> Bus Selector15/1
  AddSub281/1 -> AddSub282/2
  Delay290/1 -> Bus Creator16/15
  CMult280/1 -> AddSub283/1
  AddSub279/1 -> AddSub297/2
  Delay282/1 -> Bus Creator16/7
  Delay279/1 -> Bus Creator16/8
  CMult288/1 -> AddSub292/1
  AddSub287/1 -> AddSub295/2
  Delay293/1 -> Bus Creator16/3
  Bus Selector15/2 -> Delay283/1, CMult282/1  "<signal2>"
  CMult287/1 -> AddSub293/1
  Delay274/1 -> Bus Creator16/1
  CMult293/1 -> AddSub279/1
  Bus Selector15/19 -> CMult292/1, Delay292/1  "<signal19>"
  Delay278/1 -> Bus Creator16/5
  AddSub289/1 -> AddSub279/2
  AddSub292/1 -> AddSub293/2
  Bus Selector15/13 -> Delay286/1, CMult285/1  "<signal13>"
  Bus Selector15/10 -> CMult279/1, Delay280/1  "<signal10>"
  CMult291/1 -> AddSub287/1
  AddSub284/1 -> AddSub287/2
  CMult283/1 -> AddSub295/1
  CMult281/1 -> AddSub282/1
  Delay284/1 -> Bus Creator16/12
  Delay285/1 -> Bus Creator16/14
  Bus Selector15/12 -> Delay284/1, CMult283/1  "<signal12>"
  CMult286/1 -> AddSub294/1
  Delay288/1 -> Bus Creator16/18
  Bus Selector15/15 -> Delay290/1, CMult289/1  "<signal15>"
  Bus Selector15/9 -> Delay281/1, CMult280/1  "<signal9>"
  AddSub295/1 -> AddSub288/2
  Delay286/1 -> Bus Creator16/13
  Delay280/1 -> Bus Creator16/10
  Bus Selector15/17 -> Delay289/1, CMult288/1  "<signal17>"
  Delay277/1 -> Bus Creator16/6
  AddSub286/1 -> AddSub283/2
  Delay289/1 -> Bus Creator16/17
  Delay291/1 -> Bus Creator16/11
  Bus Selector15/14 -> Delay285/1, CMult284/1  "<signal14>"
  CMult275/1 -> AddSub297/1
  AddSub283/1 -> AddSub284/2
  Bus Selector15/16 -> Delay287/1, CMult286/1  "<signal16>"
  Bus Selector15/3 -> Delay293/1, CMult293/1  "<signal3>"
  AddSub282/1 -> AddSub286/2
  Bus Selector15/8 -> Delay279/1, CMult278/1  "<signal8>"
  CMult282/1 -> AddSub289/1
  CMult284/1 -> AddSub290/1
  Bus Selector15/1 -> Delay274/1, CMult274/1  "<signal1>"
  Bus Selector15/6 -> Delay277/1, CMult276/1  "<signal6>"
  CMult292/1 -> AddSub296/1
  Bus Selector15/18 -> CMult287/1, Delay288/1  "<signal18>"
  CMult279/1 -> AddSub284/1
  Bus Selector15/4 -> Delay275/1, CMult275/1  "<signal4>"
  AddSub288/1 -> AddSub290/2
  Delay281/1 -> Bus Creator16/9
  CMult276/1 -> AddSub281/1
  AddSub297/1 -> AddSub280/2
  Delay275/1 -> Bus Creator16/4
  AddSub294/1 -> AddSub292/2
  Delay292/1 -> Bus Creator16/19
  Bus Selector15/5 -> Delay278/1, CMult277/1  "<signal5>"
  CMult274/1 -> AddSub289/2
  CMult285/1 -> AddSub288/1
  AddSub291/1 -> AddSub294/2
  CMult278/1 -> AddSub286/1
  AddSub280/1 -> AddSub281/2
  Bus Selector15/11 -> Delay291/1, CMult291/1  "<signal11>"
  CMult297/1 -> AddSub299/1
  Delay306/1 -> Bus Creator17/16
  Delay302/1 -> Bus Creator17/2
  AddSub308/1 -> AddSub309/2
  AddSub311/1 -> AddSub314/2
  CMult309/1 -> AddSub309/1
  Bus Selector16/7 -> Delay301/1, CMult301/1  "<signal7>"
  Bus Creator16/1 -> Bus Selector16/1
  AddSub300/1 -> AddSub301/2
  Delay310/1 -> Bus Creator17/15
  CMult300/1 -> AddSub302/1
  AddSub298/1 -> AddSub315/2
  Delay301/1 -> Bus Creator17/7
  Delay298/1 -> Bus Creator17/8
  CMult308/1 -> AddSub310/1
  AddSub305/1 -> AddSub313/2
  Delay313/1 -> Bus Creator17/3
  Bus Selector16/2 -> Delay302/1, CMult302/1  "<signal2>"
  CMult307/1 -> AddSub311/1
  Delay294/1 -> Bus Creator17/1
  CMult312/1 -> AddSub298/1
  Bus Selector16/19 -> CMult311/1, Delay312/1  "<signal19>"
  Delay297/1 -> Bus Creator17/5
  AddSub307/1 -> AddSub298/2
  AddSub310/1 -> AddSub311/2
  Bus Selector16/13 -> Delay305/1, CMult305/1  "<signal13>"
  Bus Selector16/10 -> CMult299/1, Delay299/1  "<signal10>"
  CMult310/1 -> AddSub305/1
  AddSub303/1 -> AddSub305/2
  CMult303/1 -> AddSub313/1
  CMult301/1 -> AddSub301/1
  Delay303/1 -> Bus Creator17/12
  Delay304/1 -> Bus Creator17/14
  Bus Selector16/12 -> Delay303/1, CMult303/1  "<signal12>"
  CMult306/1 -> AddSub312/1
  Delay307/1 -> Bus Creator17/18
  Bus Selector16/15 -> Delay310/1, CMult309/1  "<signal15>"
  Bus Selector16/9 -> Delay300/1, CMult300/1  "<signal9>"
  AddSub313/1 -> AddSub306/2
  Delay305/1 -> Bus Creator17/13
  Delay299/1 -> Bus Creator17/10
  Bus Selector16/17 -> Delay309/1, CMult308/1  "<signal17>"
  Delay296/1 -> Bus Creator17/6
  AddSub304/1 -> AddSub302/2
  Delay309/1 -> Bus Creator17/17
  Delay311/1 -> Bus Creator17/11
  Bus Selector16/14 -> Delay304/1, CMult304/1  "<signal14>"
  CMult295/1 -> AddSub315/1
  AddSub302/1 -> AddSub303/2
  Bus Selector16/16 -> Delay306/1, CMult306/1  "<signal16>"
  Bus Selector16/3 -> Delay313/1, CMult312/1  "<signal3>"
  AddSub301/1 -> AddSub304/2
  Bus Selector16/8 -> Delay298/1, CMult298/1  "<signal8>"
  CMult302/1 -> AddSub307/1
  CMult304/1 -> AddSub308/1
  Bus Selector16/1 -> Delay294/1, CMult294/1  "<signal1>"
  Bus Selector16/6 -> Delay296/1, CMult296/1  "<signal6>"
  CMult311/1 -> AddSub314/1
  Bus Selector16/18 -> CMult307/1, Delay307/1  "<signal18>"
  CMult299/1 -> AddSub303/1
  Bus Selector16/4 -> Delay295/1, CMult295/1  "<signal4>"
  AddSub306/1 -> AddSub308/2
  Delay300/1 -> Bus Creator17/9
  CMult296/1 -> AddSub300/1
  AddSub315/1 -> AddSub299/2
  Delay295/1 -> Bus Creator17/4
  AddSub312/1 -> AddSub310/2
  Delay312/1 -> Bus Creator17/19
  Bus Selector16/5 -> Delay297/1, CMult297/1  "<signal5>"
  CMult294/1 -> AddSub307/2
  CMult305/1 -> AddSub306/1
  AddSub309/1 -> AddSub312/2
  CMult298/1 -> AddSub304/1
  AddSub299/1 -> AddSub300/2
  Bus Selector16/11 -> Delay311/1, CMult310/1  "<signal11>"
  CMult316/1 -> AddSub318/1
  Delay326/1 -> Bus Creator18/16
  Delay322/1 -> Bus Creator18/2
  AddSub328/1 -> AddSub329/2
  AddSub331/1 -> AddSub334/2
  CMult329/1 -> AddSub329/1
  Bus Selector17/7 -> Delay321/1, CMult321/1  "<signal7>"
  Bus Creator17/1 -> Bus Selector17/1
  AddSub319/1 -> AddSub320/2
  Delay329/1 -> Bus Creator18/15
  CMult319/1 -> AddSub321/1
  AddSub317/1 -> AddSub335/2
  Delay321/1 -> Bus Creator18/7
  Delay318/1 -> Bus Creator18/8
  CMult328/1 -> AddSub330/1
  AddSub325/1 -> AddSub333/2
  Delay332/1 -> Bus Creator18/3
  Bus Selector17/2 -> Delay322/1, CMult322/1  "<signal2>"
  CMult327/1 -> AddSub331/1
  Delay314/1 -> Bus Creator18/1
  CMult332/1 -> AddSub317/1
  Bus Selector17/19 -> CMult331/1, Delay331/1  "<signal19>"
  Delay317/1 -> Bus Creator18/5
  AddSub327/1 -> AddSub317/2
  AddSub330/1 -> AddSub331/2
  Bus Selector17/13 -> Delay325/1, CMult325/1  "<signal13>"
  Bus Selector17/10 -> CMult318/1, Delay319/1  "<signal10>"
  CMult330/1 -> AddSub325/1
  AddSub322/1 -> AddSub325/2
  CMult323/1 -> AddSub333/1
  CMult321/1 -> AddSub320/1
  Delay323/1 -> Bus Creator18/12
  Delay324/1 -> Bus Creator18/14
  Bus Selector17/12 -> Delay323/1, CMult323/1  "<signal12>"
  CMult326/1 -> AddSub332/1
  Delay327/1 -> Bus Creator18/18
  Bus Selector17/15 -> Delay329/1, CMult329/1  "<signal15>"
  Bus Selector17/9 -> Delay320/1, CMult319/1  "<signal9>"
  AddSub333/1 -> AddSub326/2
  Delay325/1 -> Bus Creator18/13
  Delay319/1 -> Bus Creator18/10
  Bus Selector17/17 -> Delay328/1, CMult328/1  "<signal17>"
  Delay316/1 -> Bus Creator18/6
  AddSub323/1 -> AddSub321/2
  Delay328/1 -> Bus Creator18/17
  Delay330/1 -> Bus Creator18/11
  Bus Selector17/14 -> Delay324/1, CMult324/1  "<signal14>"
  CMult314/1 -> AddSub335/1
  AddSub321/1 -> AddSub322/2
  Bus Selector17/16 -> Delay326/1, CMult326/1  "<signal16>"
  Bus Selector17/3 -> Delay332/1, CMult332/1  "<signal3>"
  AddSub320/1 -> AddSub323/2
  Bus Selector17/8 -> Delay318/1, CMult317/1  "<signal8>"
  CMult322/1 -> AddSub327/1
  CMult324/1 -> AddSub328/1
  Bus Selector17/1 -> Delay314/1, CMult313/1  "<signal1>"
  Bus Selector17/6 -> Delay316/1, CMult315/1  "<signal6>"
  CMult331/1 -> AddSub334/1
  Bus Selector17/18 -> CMult327/1, Delay327/1  "<signal18>"
  CMult318/1 -> AddSub322/1
  Bus Selector17/4 -> Delay315/1, CMult314/1  "<signal4>"
  AddSub326/1 -> AddSub328/2
  Delay320/1 -> Bus Creator18/9
  CMult315/1 -> AddSub319/1
  AddSub335/1 -> AddSub318/2
  Delay315/1 -> Bus Creator18/4
  AddSub332/1 -> AddSub330/2
  Delay331/1 -> Bus Creator18/19
  Bus Selector17/5 -> Delay317/1, CMult316/1  "<signal5>"
  CMult313/1 -> AddSub327/2
  CMult325/1 -> AddSub326/1
  AddSub329/1 -> AddSub332/2
  CMult317/1 -> AddSub323/1
  AddSub318/1 -> AddSub319/2
  Bus Selector17/11 -> Delay330/1, CMult330/1  "<signal11>"
  CMult336/1 -> AddSub337/1
  Delay346/1 -> Bus Creator19/16
  Delay341/1 -> Bus Creator19/2
  AddSub346/1 -> AddSub347/2
  AddSub349/1 -> AddSub352/2
  CMult348/1 -> AddSub347/1
  Bus Selector18/7 -> Delay340/1, CMult340/1  "<signal7>"
  Bus Creator18/1 -> Bus Selector18/1
  AddSub338/1 -> AddSub339/2
  Delay349/1 -> Bus Creator19/15
  CMult339/1 -> AddSub340/1
  AddSub336/1 -> AddSub353/2
  Delay340/1 -> Bus Creator19/7
  Delay337/1 -> Bus Creator19/8
  CMult347/1 -> AddSub348/1
  AddSub343/1 -> AddSub351/2
  Delay352/1 -> Bus Creator19/3
  Bus Selector18/2 -> Delay341/1, CMult341/1  "<signal2>"
  CMult346/1 -> AddSub349/1
  Delay333/1 -> Bus Creator19/1
  CMult351/1 -> AddSub336/1
  Bus Selector18/19 -> CMult350/1, Delay351/1  "<signal19>"
  Delay336/1 -> Bus Creator19/5
  AddSub345/1 -> AddSub336/2
  AddSub348/1 -> AddSub349/2
  Bus Selector18/13 -> Delay345/1, CMult344/1  "<signal13>"
  Bus Selector18/10 -> CMult338/1, Delay338/1  "<signal10>"
  CMult349/1 -> AddSub343/1
  AddSub341/1 -> AddSub343/2
  CMult342/1 -> AddSub351/1
  CMult340/1 -> AddSub339/1
  Delay342/1 -> Bus Creator19/12
  Delay343/1 -> Bus Creator19/14
  Bus Selector18/12 -> Delay342/1, CMult342/1  "<signal12>"
  CMult345/1 -> AddSub350/1
  Delay347/1 -> Bus Creator19/18
  Bus Selector18/15 -> Delay349/1, CMult348/1  "<signal15>"
  Bus Selector18/9 -> Delay339/1, CMult339/1  "<signal9>"
  AddSub351/1 -> AddSub344/2
  Delay345/1 -> Bus Creator19/13
  Delay338/1 -> Bus Creator19/10
  Bus Selector18/17 -> Delay348/1, CMult347/1  "<signal17>"
  Delay335/1 -> Bus Creator19/6
  AddSub342/1 -> AddSub340/2
  Delay348/1 -> Bus Creator19/17
  Delay350/1 -> Bus Creator19/11
  Bus Selector18/14 -> Delay343/1, CMult343/1  "<signal14>"
  CMult334/1 -> AddSub353/1
  AddSub340/1 -> AddSub341/2
  Bus Selector18/16 -> Delay346/1, CMult345/1  "<signal16>"
  Bus Selector18/3 -> Delay352/1, CMult351/1  "<signal3>"
  AddSub339/1 -> AddSub342/2
  Bus Selector18/8 -> Delay337/1, CMult337/1  "<signal8>"
  CMult341/1 -> AddSub345/1
  CMult343/1 -> AddSub346/1
  Bus Selector18/1 -> Delay333/1, CMult333/1  "<signal1>"
  Bus Selector18/6 -> Delay335/1, CMult335/1  "<signal6>"
  CMult350/1 -> AddSub352/1
  Bus Selector18/18 -> CMult346/1, Delay347/1  "<signal18>"
  CMult338/1 -> AddSub341/1
  Bus Selector18/4 -> Delay334/1, CMult334/1  "<signal4>"
  AddSub344/1 -> AddSub346/2
  Delay339/1 -> Bus Creator19/9
  CMult335/1 -> AddSub338/1
  AddSub353/1 -> AddSub337/2
  Delay334/1 -> Bus Creator19/4
  AddSub350/1 -> AddSub348/2
  Delay351/1 -> Bus Creator19/19
  Bus Selector18/5 -> Delay336/1, CMult336/1  "<signal5>"
  CMult333/1 -> AddSub345/2
  CMult344/1 -> AddSub344/1
  AddSub347/1 -> AddSub350/2
  CMult337/1 -> AddSub342/1
  AddSub337/1 -> AddSub338/2
  Bus Selector18/11 -> Delay350/1, CMult349/1  "<signal11>"
